simulink model "fft_4ch_nofir"  (R2012b)
settings: Solver=FixedStepDiscrete  SolverMode=SingleTasking  StartTime=0.0  StopTime=32768*5  FixedStep=0.25  RelTol=1e-3
libraries: xbsIndex_r4 x17003, casper_library_misc x133, casper_library_multipliers x20, casper_library_delays x19, xps_library x5, dspsrcs4 x3, xbsReplacements_r4 x2, simulink x1
(part 3 of 170)

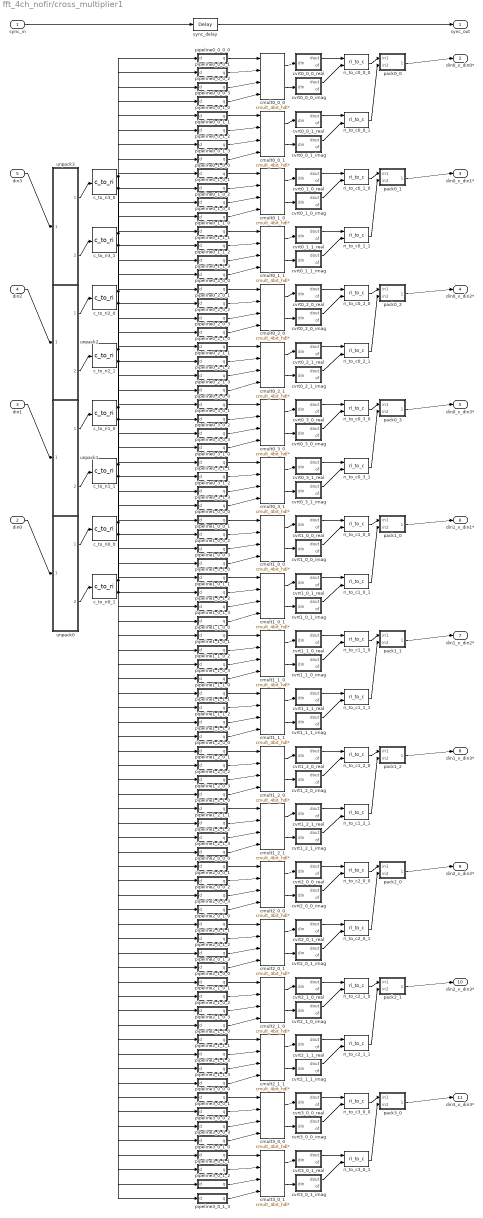
== system fft_4ch_nofir/cross_multiplier1 ==
  sync_in : Inport
  din0 : Inport  Port=2
  din1 : Inport  Port=3
  din2 : Inport  Port=4
  din3 : Inport  Port=5
  c_to_ri0_0 : casper_library_misc/c_to_ri  n_bits=bit_width_in  bin_pt=binary_point_in
  c_to_ri0_1 : casper_library_misc/c_to_ri  n_bits=bit_width_in  bin_pt=binary_point_in
  c_to_ri1_0 : casper_library_misc/c_to_ri  n_bits=bit_width_in  bin_pt=binary_point_in
  c_to_ri1_1 : casper_library_misc/c_to_ri  n_bits=bit_width_in  bin_pt=binary_point_in
  c_to_ri2_0 : casper_library_misc/c_to_ri  n_bits=bit_width_in  bin_pt=binary_point_in
  c_to_ri2_1 : casper_library_misc/c_to_ri  n_bits=bit_width_in  bin_pt=binary_point_in
  c_to_ri3_0 : casper_library_misc/c_to_ri  n_bits=bit_width_in  bin_pt=binary_point_in
  c_to_ri3_1 : casper_library_misc/c_to_ri  n_bits=bit_width_in  bin_pt=binary_point_in
  cmult0_0_0 : casper_library_multipliers/cmult_4bit_hdl*  mult_latency=mult_latency  add_latency=add_latency
      link override imag_sum: mode=Subtraction  use_carryin=off  use_carryout=off  en=off  latency=add_latency  precision=Full  arith_type=Unsigned  n_bits=8  bin_pt=2  quantization=Truncate  overflow=Wrap  dbl_ovrd=off  use_behavioral_HDL=on  hw_selection=Fabric  pipelined=off  use_rpm=on
      link override real_sum: mode=Addition  use_carryin=off  use_carryout=off  en=off  latency=add_latency  precision=Full  arith_type=Unsigned  n_bits=8  bin_pt=2  quantization=Truncate  overflow=Wrap  dbl_ovrd=off  use_behavioral_HDL=on  hw_selection=Fabric  pipelined=off  use_rpm=on
      link override imag_sum: xl_area=[4 8 0 7 0 0 0]
      link override real_sum: xl_area=[4 8 0 7 0 0 0]
  cmult0_0_1 : casper_library_multipliers/cmult_4bit_hdl*  mult_latency=mult_latency  add_latency=add_latency
  cmult0_1_0 : casper_library_multipliers/cmult_4bit_hdl*  mult_latency=mult_latency  add_latency=add_latency
  cmult0_1_1 : casper_library_multipliers/cmult_4bit_hdl*  mult_latency=mult_latency  add_latency=add_latency
  cmult0_2_0 : casper_library_multipliers/cmult_4bit_hdl*  mult_latency=mult_latency  add_latency=add_latency
  cmult0_2_1 : casper_library_multipliers/cmult_4bit_hdl*  mult_latency=mult_latency  add_latency=add_latency
  cmult0_3_0 : casper_library_multipliers/cmult_4bit_hdl*  mult_latency=mult_latency  add_latency=add_latency
  cmult0_3_1 : casper_library_multipliers/cmult_4bit_hdl*  mult_latency=mult_latency  add_latency=add_latency
  cmult1_0_0 : casper_library_multipliers/cmult_4bit_hdl*  mult_latency=mult_latency  add_latency=add_latency
  cmult1_0_1 : casper_library_multipliers/cmult_4bit_hdl*  mult_latency=mult_latency  add_latency=add_latency
  cmult1_1_0 : casper_library_multipliers/cmult_4bit_hdl*  mult_latency=mult_latency  add_latency=add_latency
  cmult1_1_1 : casper_library_multipliers/cmult_4bit_hdl*  mult_latency=mult_latency  add_latency=add_latency
  cmult1_2_0 : casper_library_multipliers/cmult_4bit_hdl*  mult_latency=mult_latency  add_latency=add_latency
  cmult1_2_1 : casper_library_multipliers/cmult_4bit_hdl*  mult_latency=mult_latency  add_latency=add_latency
  cmult2_0_0 : casper_library_multipliers/cmult_4bit_hdl*  mult_latency=mult_latency  add_latency=add_latency
  cmult2_0_1 : casper_library_multipliers/cmult_4bit_hdl*  mult_latency=mult_latency  add_latency=add_latency
  cmult2_1_0 : casper_library_multipliers/cmult_4bit_hdl*  mult_latency=mult_latency  add_latency=add_latency
  cmult2_1_1 : casper_library_multipliers/cmult_4bit_hdl*  mult_latency=mult_latency  add_latency=add_latency
  cmult3_0_0 : casper_library_multipliers/cmult_4bit_hdl*  mult_latency=mult_latency  add_latency=add_latency
  cmult3_0_1 : casper_library_multipliers/cmult_4bit_hdl*  mult_latency=mult_latency  add_latency=add_latency
  cvrt0_0_0_imag : Subsystem  AncestorBlock=casper_library_misc/convert_of  mask(convert_of){bit_width_i=37, binary_point_i=34, bit_width_o=37, binary_point_o=34, latency=0, overflow=Wrap, quantization=Truncate}
      mask prompts: bit_width_i "Bit Width In"; binary_point_i "Binary Point In"; bit_width_o "Bit Width Out"; binary_point_o "Binary Point Out"; overflow "Overflow Behaviour"; quantization "Quantization Behaviour"
      mask help:
      | Converts from one 2's complement bit-width
      | and/or binary point position to another.
      | Includes underflow/overflow indicator.
      mask init:
      | convert_of_init(gcb, ...
      |     'bit_width_i', bit_width_i, ...
      |     'binary_point_i', binary_point_i, ...
      |     'bit_width_o', bit_width_o, ...
      |     'binary_point_o', binary_point_o, ...
      |     'latency', latency, ...
      |     'overflow', overflow, ...
      |     'quantization', quantization);
      settings: AttributesFormatString=[37,34]->[37,34]
      mask TypeOptions overflow: Wrap | Saturate | Error
      mask TypeOptions quantization: Truncate | Round  (unbiased: +/- Inf) | Round  (unbiased: even values)
  cvrt0_0_0_real : Subsystem  AncestorBlock=casper_library_misc/convert_of  mask(convert_of){bit_width_i=37, binary_point_i=34, bit_width_o=37, binary_point_o=34, latency=0, overflow=Wrap, quantization=Truncate}
      mask prompts: bit_width_i "Bit Width In"; binary_point_i "Binary Point In"; bit_width_o "Bit Width Out"; binary_point_o "Binary Point Out"; overflow "Overflow Behaviour"; quantization "Quantization Behaviour"
      mask help:
      | Converts from one 2's complement bit-width
      | and/or binary point position to another.
      | Includes underflow/overflow indicator.
      mask init: same as fft_4ch_nofir/cross_multiplier1/cvrt0_0_0_imag
      settings: AttributesFormatString=[37,34]->[37,34]
      mask TypeOptions overflow: Wrap | Saturate | Error
      mask TypeOptions quantization: Truncate | Round  (unbiased: +/- Inf) | Round  (unbiased: even values)
  cvrt0_0_1_imag : Subsystem  AncestorBlock=casper_library_misc/convert_of  mask(convert_of){bit_width_i=37, binary_point_i=34, bit_width_o=37, binary_point_o=34, latency=0, overflow=Wrap, quantization=Truncate}
      mask prompts: bit_width_i "Bit Width In"; binary_point_i "Binary Point In"; bit_width_o "Bit Width Out"; binary_point_o "Binary Point Out"; overflow "Overflow Behaviour"; quantization "Quantization Behaviour"
      mask help:
      | Converts from one 2's complement bit-width
      | and/or binary point position to another.
      | Includes underflow/overflow indicator.
      mask init: same as fft_4ch_nofir/cross_multiplier1/cvrt0_0_0_imag
      settings: AttributesFormatString=[37,34]->[37,34]
      mask TypeOptions overflow: Wrap | Saturate | Error
      mask TypeOptions quantization: Truncate | Round  (unbiased: +/- Inf) | Round  (unbiased: even values)
  cvrt0_0_1_real : Subsystem  AncestorBlock=casper_library_misc/convert_of  mask(convert_of){bit_width_i=37, binary_point_i=34, bit_width_o=37, binary_point_o=34, latency=0, overflow=Wrap, quantization=Truncate}
      mask prompts: bit_width_i "Bit Width In"; binary_point_i "Binary Point In"; bit_width_o "Bit Width Out"; binary_point_o "Binary Point Out"; overflow "Overflow Behaviour"; quantization "Quantization Behaviour"
      mask help:
      | Converts from one 2's complement bit-width
      | and/or binary point position to another.
      | Includes underflow/overflow indicator.
      mask init: same as fft_4ch_nofir/cross_multiplier1/cvrt0_0_0_imag
      settings: AttributesFormatString=[37,34]->[37,34]
      mask TypeOptions overflow: Wrap | Saturate | Error
      mask TypeOptions quantization: Truncate | Round  (unbiased: +/- Inf) | Round  (unbiased: even values)
  cvrt0_1_0_imag : Subsystem  AncestorBlock=casper_library_misc/convert_of  mask(convert_of){bit_width_i=37, binary_point_i=34, bit_width_o=37, binary_point_o=34, latency=0, overflow=Wrap, quantization=Truncate}
      mask prompts: bit_width_i "Bit Width In"; binary_point_i "Binary Point In"; bit_width_o "Bit Width Out"; binary_point_o "Binary Point Out"; overflow "Overflow Behaviour"; quantization "Quantization Behaviour"
      mask help:
      | Converts from one 2's complement bit-width
      | and/or binary point position to another.
      | Includes underflow/overflow indicator.
      mask init: same as fft_4ch_nofir/cross_multiplier1/cvrt0_0_0_imag
      settings: AttributesFormatString=[37,34]->[37,34]
      mask TypeOptions overflow: Wrap | Saturate | Error
      mask TypeOptions quantization: Truncate | Round  (unbiased: +/- Inf) | Round  (unbiased: even values)
  cvrt0_1_0_real : Subsystem  AncestorBlock=casper_library_misc/convert_of  mask(convert_of){bit_width_i=37, binary_point_i=34, bit_width_o=37, binary_point_o=34, latency=0, overflow=Wrap, quantization=Truncate}
      mask prompts: bit_width_i "Bit Width In"; binary_point_i "Binary Point In"; bit_width_o "Bit Width Out"; binary_point_o "Binary Point Out"; overflow "Overflow Behaviour"; quantization "Quantization Behaviour"
      mask help:
      | Converts from one 2's complement bit-width
      | and/or binary point position to another.
      | Includes underflow/overflow indicator.
      mask init: same as fft_4ch_nofir/cross_multiplier1/cvrt0_0_0_imag
      settings: AttributesFormatString=[37,34]->[37,34]
      mask TypeOptions overflow: Wrap | Saturate | Error
      mask TypeOptions quantization: Truncate | Round  (unbiased: +/- Inf) | Round  (unbiased: even values)
  cvrt0_1_1_imag : Subsystem  AncestorBlock=casper_library_misc/convert_of  mask(convert_of){bit_width_i=37, binary_point_i=34, bit_width_o=37, binary_point_o=34, latency=0, overflow=Wrap, quantization=Truncate}
      mask prompts: bit_width_i "Bit Width In"; binary_point_i "Binary Point In"; bit_width_o "Bit Width Out"; binary_point_o "Binary Point Out"; overflow "Overflow Behaviour"; quantization "Quantization Behaviour"
      mask help:
      | Converts from one 2's complement bit-width
      | and/or binary point position to another.
      | Includes underflow/overflow indicator.
      mask init: same as fft_4ch_nofir/cross_multiplier1/cvrt0_0_0_imag
      settings: AttributesFormatString=[37,34]->[37,34]
      mask TypeOptions overflow: Wrap | Saturate | Error
      mask TypeOptions quantization: Truncate | Round  (unbiased: +/- Inf) | Round  (unbiased: even values)
  cvrt0_1_1_real : Subsystem  AncestorBlock=casper_library_misc/convert_of  mask(convert_of){bit_width_i=37, binary_point_i=34, bit_width_o=37, binary_point_o=34, latency=0, overflow=Wrap, quantization=Truncate}
      mask prompts: bit_width_i "Bit Width In"; binary_point_i "Binary Point In"; bit_width_o "Bit Width Out"; binary_point_o "Binary Point Out"; overflow "Overflow Behaviour"; quantization "Quantization Behaviour"
      mask help:
      | Converts from one 2's complement bit-width
      | and/or binary point position to another.
      | Includes underflow/overflow indicator.
      mask init: same as fft_4ch_nofir/cross_multiplier1/cvrt0_0_0_imag
      settings: AttributesFormatString=[37,34]->[37,34]
      mask TypeOptions overflow: Wrap | Saturate | Error
      mask TypeOptions quantization: Truncate | Round  (unbiased: +/- Inf) | Round  (unbiased: even values)
  cvrt0_2_0_imag : Subsystem  AncestorBlock=casper_library_misc/convert_of  mask(convert_of){bit_width_i=37, binary_point_i=34, bit_width_o=37, binary_point_o=34, latency=0, overflow=Wrap, quantization=Truncate}
      mask prompts: bit_width_i "Bit Width In"; binary_point_i "Binary Point In"; bit_width_o "Bit Width Out"; binary_point_o "Binary Point Out"; overflow "Overflow Behaviour"; quantization "Quantization Behaviour"
      mask help:
      | Converts from one 2's complement bit-width
      | and/or binary point position to another.
      | Includes underflow/overflow indicator.
      mask init: same as fft_4ch_nofir/cross_multiplier1/cvrt0_0_0_imag
      settings: AttributesFormatString=[37,34]->[37,34]
      mask TypeOptions overflow: Wrap | Saturate | Error
      mask TypeOptions quantization: Truncate | Round  (unbiased: +/- Inf) | Round  (unbiased: even values)
  cvrt0_2_0_real : Subsystem  AncestorBlock=casper_library_misc/convert_of  mask(convert_of){bit_width_i=37, binary_point_i=34, bit_width_o=37, binary_point_o=34, latency=0, overflow=Wrap, quantization=Truncate}
      mask prompts: bit_width_i "Bit Width In"; binary_point_i "Binary Point In"; bit_width_o "Bit Width Out"; binary_point_o "Binary Point Out"; overflow "Overflow Behaviour"; quantization "Quantization Behaviour"
      mask help:
      | Converts from one 2's complement bit-width
      | and/or binary point position to another.
      | Includes underflow/overflow indicator.
      mask init: same as fft_4ch_nofir/cross_multiplier1/cvrt0_0_0_imag
      settings: AttributesFormatString=[37,34]->[37,34]
      mask TypeOptions overflow: Wrap | Saturate | Error
      mask TypeOptions quantization: Truncate | Round  (unbiased: +/- Inf) | Round  (unbiased: even values)
  cvrt0_2_1_imag : Subsystem  AncestorBlock=casper_library_misc/convert_of  mask(convert_of){bit_width_i=37, binary_point_i=34, bit_width_o=37, binary_point_o=34, latency=0, overflow=Wrap, quantization=Truncate}
      mask prompts: bit_width_i "Bit Width In"; binary_point_i "Binary Point In"; bit_width_o "Bit Width Out"; binary_point_o "Binary Point Out"; overflow "Overflow Behaviour"; quantization "Quantization Behaviour"
      mask help:
      | Converts from one 2's complement bit-width
      | and/or binary point position to another.
      | Includes underflow/overflow indicator.
      mask init: same as fft_4ch_nofir/cross_multiplier1/cvrt0_0_0_imag
      settings: AttributesFormatString=[37,34]->[37,34]
      mask TypeOptions overflow: Wrap | Saturate | Error
      mask TypeOptions quantization: Truncate | Round  (unbiased: +/- Inf) | Round  (unbiased: even values)
  cvrt0_2_1_real : Subsystem  AncestorBlock=casper_library_misc/convert_of  mask(convert_of){bit_width_i=37, binary_point_i=34, bit_width_o=37, binary_point_o=34, latency=0, overflow=Wrap, quantization=Truncate}
      mask prompts: bit_width_i "Bit Width In"; binary_point_i "Binary Point In"; bit_width_o "Bit Width Out"; binary_point_o "Binary Point Out"; overflow "Overflow Behaviour"; quantization "Quantization Behaviour"
      mask help:
      | Converts from one 2's complement bit-width
      | and/or binary point position to another.
      | Includes underflow/overflow indicator.
      mask init: same as fft_4ch_nofir/cross_multiplier1/cvrt0_0_0_imag
      settings: AttributesFormatString=[37,34]->[37,34]
      mask TypeOptions overflow: Wrap | Saturate | Error
      mask TypeOptions quantization: Truncate | Round  (unbiased: +/- Inf) | Round  (unbiased: even values)
  cvrt0_3_0_imag : Subsystem  AncestorBlock=casper_library_misc/convert_of  mask(convert_of){bit_width_i=37, binary_point_i=34, bit_width_o=37, binary_point_o=34, latency=0, overflow=Wrap, quantization=Truncate}
      mask prompts: bit_width_i "Bit Width In"; binary_point_i "Binary Point In"; bit_width_o "Bit Width Out"; binary_point_o "Binary Point Out"; overflow "Overflow Behaviour"; quantization "Quantization Behaviour"
      mask help:
      | Converts from one 2's complement bit-width
      | and/or binary point position to another.
      | Includes underflow/overflow indicator.
      mask init: same as fft_4ch_nofir/cross_multiplier1/cvrt0_0_0_imag
      settings: AttributesFormatString=[37,34]->[37,34]
      mask TypeOptions overflow: Wrap | Saturate | Error
      mask TypeOptions quantization: Truncate | Round  (unbiased: +/- Inf) | Round  (unbiased: even values)
  cvrt0_3_0_real : Subsystem  AncestorBlock=casper_library_misc/convert_of  mask(convert_of){bit_width_i=37, binary_point_i=34, bit_width_o=37, binary_point_o=34, latency=0, overflow=Wrap, quantization=Truncate}
      mask prompts: bit_width_i "Bit Width In"; binary_point_i "Binary Point In"; bit_width_o "Bit Width Out"; binary_point_o "Binary Point Out"; overflow "Overflow Behaviour"; quantization "Quantization Behaviour"
      mask help:
      | Converts from one 2's complement bit-width
      | and/or binary point position to another.
      | Includes underflow/overflow indicator.
      mask init: same as fft_4ch_nofir/cross_multiplier1/cvrt0_0_0_imag
      settings: AttributesFormatString=[37,34]->[37,34]
      mask TypeOptions overflow: Wrap | Saturate | Error
      mask TypeOptions quantization: Truncate | Round  (unbiased: +/- Inf) | Round  (unbiased: even values)
  cvrt0_3_1_imag : Subsystem  AncestorBlock=casper_library_misc/convert_of  mask(convert_of){bit_width_i=37, binary_point_i=34, bit_width_o=37, binary_point_o=34, latency=0, overflow=Wrap, quantization=Truncate}
      mask prompts: bit_width_i "Bit Width In"; binary_point_i "Binary Point In"; bit_width_o "Bit Width Out"; binary_point_o "Binary Point Out"; overflow "Overflow Behaviour"; quantization "Quantization Behaviour"
      mask help:
      | Converts from one 2's complement bit-width
      | and/or binary point position to another.
      | Includes underflow/overflow indicator.
      mask init: same as fft_4ch_nofir/cross_multiplier1/cvrt0_0_0_imag
      settings: AttributesFormatString=[37,34]->[37,34]
      mask TypeOptions overflow: Wrap | Saturate | Error
      mask TypeOptions quantization: Truncate | Round  (unbiased: +/- Inf) | Round  (unbiased: even values)
  cvrt0_3_1_real : Subsystem  AncestorBlock=casper_library_misc/convert_of  mask(convert_of){bit_width_i=37, binary_point_i=34, bit_width_o=37, binary_point_o=34, latency=0, overflow=Wrap, quantization=Truncate}
      mask prompts: bit_width_i "Bit Width In"; binary_point_i "Binary Point In"; bit_width_o "Bit Width Out"; binary_point_o "Binary Point Out"; overflow "Overflow Behaviour"; quantization "Quantization Behaviour"
      mask help:
      | Converts from one 2's complement bit-width
      | and/or binary point position to another.
      | Includes underflow/overflow indicator.
      mask init: same as fft_4ch_nofir/cross_multiplier1/cvrt0_0_0_imag
      settings: AttributesFormatString=[37,34]->[37,34]
      mask TypeOptions overflow: Wrap | Saturate | Error
      mask TypeOptions quantization: Truncate | Round  (unbiased: +/- Inf) | Round  (unbiased: even values)
  cvrt1_0_0_imag : Subsystem  AncestorBlock=casper_library_misc/convert_of  mask(convert_of){bit_width_i=37, binary_point_i=34, bit_width_o=37, binary_point_o=34, latency=0, overflow=Wrap, quantization=Truncate}
      mask prompts: bit_width_i "Bit Width In"; binary_point_i "Binary Point In"; bit_width_o "Bit Width Out"; binary_point_o "Binary Point Out"; overflow "Overflow Behaviour"; quantization "Quantization Behaviour"
      mask help:
      | Converts from one 2's complement bit-width
      | and/or binary point position to another.
      | Includes underflow/overflow indicator.
      mask init: same as fft_4ch_nofir/cross_multiplier1/cvrt0_0_0_imag
      settings: AttributesFormatString=[37,34]->[37,34]
      mask TypeOptions overflow: Wrap | Saturate | Error
      mask TypeOptions quantization: Truncate | Round  (unbiased: +/- Inf) | Round  (unbiased: even values)
  cvrt1_0_0_real : Subsystem  AncestorBlock=casper_library_misc/convert_of  mask(convert_of){bit_width_i=37, binary_point_i=34, bit_width_o=37, binary_point_o=34, latency=0, overflow=Wrap, quantization=Truncate}
      mask prompts: bit_width_i "Bit Width In"; binary_point_i "Binary Point In"; bit_width_o "Bit Width Out"; binary_point_o "Binary Point Out"; overflow "Overflow Behaviour"; quantization "Quantization Behaviour"
      mask help:
      | Converts from one 2's complement bit-width
      | and/or binary point position to another.
      | Includes underflow/overflow indicator.
      mask init: same as fft_4ch_nofir/cross_multiplier1/cvrt0_0_0_imag
      settings: AttributesFormatString=[37,34]->[37,34]
      mask TypeOptions overflow: Wrap | Saturate | Error
      mask TypeOptions quantization: Truncate | Round  (unbiased: +/- Inf) | Round  (unbiased: even values)
  cvrt1_0_1_imag : Subsystem  AncestorBlock=casper_library_misc/convert_of  mask(convert_of){bit_width_i=37, binary_point_i=34, bit_width_o=37, binary_point_o=34, latency=0, overflow=Wrap, quantization=Truncate}
      mask prompts: bit_width_i "Bit Width In"; binary_point_i "Binary Point In"; bit_width_o "Bit Width Out"; binary_point_o "Binary Point Out"; overflow "Overflow Behaviour"; quantization "Quantization Behaviour"
      mask help:
      | Converts from one 2's complement bit-width
      | and/or binary point position to another.
      | Includes underflow/overflow indicator.
      mask init: same as fft_4ch_nofir/cross_multiplier1/cvrt0_0_0_imag
      settings: AttributesFormatString=[37,34]->[37,34]
      mask TypeOptions overflow: Wrap | Saturate | Error
      mask TypeOptions quantization: Truncate | Round  (unbiased: +/- Inf) | Round  (unbiased: even values)
  cvrt1_0_1_real : Subsystem  AncestorBlock=casper_library_misc/convert_of  mask(convert_of){bit_width_i=37, binary_point_i=34, bit_width_o=37, binary_point_o=34, latency=0, overflow=Wrap, quantization=Truncate}
      mask prompts: bit_width_i "Bit Width In"; binary_point_i "Binary Point In"; bit_width_o "Bit Width Out"; binary_point_o "Binary Point Out"; overflow "Overflow Behaviour"; quantization "Quantization Behaviour"
      mask help:
      | Converts from one 2's complement bit-width
      | and/or binary point position to another.
      | Includes underflow/overflow indicator.
      mask init: same as fft_4ch_nofir/cross_multiplier1/cvrt0_0_0_imag
      settings: AttributesFormatString=[37,34]->[37,34]
      mask TypeOptions overflow: Wrap | Saturate | Error
      mask TypeOptions quantization: Truncate | Round  (unbiased: +/- Inf) | Round  (unbiased: even values)
  cvrt1_1_0_imag : Subsystem  AncestorBlock=casper_library_misc/convert_of  mask(convert_of){bit_width_i=37, binary_point_i=34, bit_width_o=37, binary_point_o=34, latency=0, overflow=Wrap, quantization=Truncate}
      mask prompts: bit_width_i "Bit Width In"; binary_point_i "Binary Point In"; bit_width_o "Bit Width Out"; binary_point_o "Binary Point Out"; overflow "Overflow Behaviour"; quantization "Quantization Behaviour"
      mask help:
      | Converts from one 2's complement bit-width
      | and/or binary point position to another.
      | Includes underflow/overflow indicator.
      mask init: same as fft_4ch_nofir/cross_multiplier1/cvrt0_0_0_imag
      settings: AttributesFormatString=[37,34]->[37,34]
      mask TypeOptions overflow: Wrap | Saturate | Error
      mask TypeOptions quantization: Truncate | Round  (unbiased: +/- Inf) | Round  (unbiased: even values)
  cvrt1_1_0_real : Subsystem  AncestorBlock=casper_library_misc/convert_of  mask(convert_of){bit_width_i=37, binary_point_i=34, bit_width_o=37, binary_point_o=34, latency=0, overflow=Wrap, quantization=Truncate}
      mask prompts: bit_width_i "Bit Width In"; binary_point_i "Binary Point In"; bit_width_o "Bit Width Out"; binary_point_o "Binary Point Out"; overflow "Overflow Behaviour"; quantization "Quantization Behaviour"
      mask help:
      | Converts from one 2's complement bit-width
      | and/or binary point position to another.
      | Includes underflow/overflow indicator.
      mask init: same as fft_4ch_nofir/cross_multiplier1/cvrt0_0_0_imag
      settings: AttributesFormatString=[37,34]->[37,34]
      mask TypeOptions overflow: Wrap | Saturate | Error
      mask TypeOptions quantization: Truncate | Round  (unbiased: +/- Inf) | Round  (unbiased: even values)
  cvrt1_1_1_imag : Subsystem  AncestorBlock=casper_library_misc/convert_of  mask(convert_of){bit_width_i=37, binary_point_i=34, bit_width_o=37, binary_point_o=34, latency=0, overflow=Wrap, quantization=Truncate}
      mask prompts: bit_width_i "Bit Width In"; binary_point_i "Binary Point In"; bit_width_o "Bit Width Out"; binary_point_o "Binary Point Out"; overflow "Overflow Behaviour"; quantization "Quantization Behaviour"
      mask help:
      | Converts from one 2's complement bit-width
      | and/or binary point position to another.
      | Includes underflow/overflow indicator.
      mask init: same as fft_4ch_nofir/cross_multiplier1/cvrt0_0_0_imag
      settings: AttributesFormatString=[37,34]->[37,34]
      mask TypeOptions overflow: Wrap | Saturate | Error
      mask TypeOptions quantization: Truncate | Round  (unbiased: +/- Inf) | Round  (unbiased: even values)
  cvrt1_1_1_real : Subsystem  AncestorBlock=casper_library_misc/convert_of  mask(convert_of){bit_width_i=37, binary_point_i=34, bit_width_o=37, binary_point_o=34, latency=0, overflow=Wrap, quantization=Truncate}
      mask prompts: bit_width_i "Bit Width In"; binary_point_i "Binary Point In"; bit_width_o "Bit Width Out"; binary_point_o "Binary Point Out"; overflow "Overflow Behaviour"; quantization "Quantization Behaviour"
      mask help:
      | Converts from one 2's complement bit-width
      | and/or binary point position to another.
      | Includes underflow/overflow indicator.
      mask init: same as fft_4ch_nofir/cross_multiplier1/cvrt0_0_0_imag
      settings: AttributesFormatString=[37,34]->[37,34]
      mask TypeOptions overflow: Wrap | Saturate | Error
      mask TypeOptions quantization: Truncate | Round  (unbiased: +/- Inf) | Round  (unbiased: even values)
  cvrt1_2_0_imag : Subsystem  AncestorBlock=casper_library_misc/convert_of  mask(convert_of){bit_width_i=37, binary_point_i=34, bit_width_o=37, binary_point_o=34, latency=0, overflow=Wrap, quantization=Truncate}
      mask prompts: bit_width_i "Bit Width In"; binary_point_i "Binary Point In"; bit_width_o "Bit Width Out"; binary_point_o "Binary Point Out"; overflow "Overflow Behaviour"; quantization "Quantization Behaviour"
      mask help:
      | Converts from one 2's complement bit-width
      | and/or binary point position to another.
      | Includes underflow/overflow indicator.
      mask init: same as fft_4ch_nofir/cross_multiplier1/cvrt0_0_0_imag
      settings: AttributesFormatString=[37,34]->[37,34]
      mask TypeOptions overflow: Wrap | Saturate | Error
      mask TypeOptions quantization: Truncate | Round  (unbiased: +/- Inf) | Round  (unbiased: even values)
  cvrt1_2_0_real : Subsystem  AncestorBlock=casper_library_misc/convert_of  mask(convert_of){bit_width_i=37, binary_point_i=34, bit_width_o=37, binary_point_o=34, latency=0, overflow=Wrap, quantization=Truncate}
      mask prompts: bit_width_i "Bit Width In"; binary_point_i "Binary Point In"; bit_width_o "Bit Width Out"; binary_point_o "Binary Point Out"; overflow "Overflow Behaviour"; quantization "Quantization Behaviour"
      mask help:
      | Converts from one 2's complement bit-width
      | and/or binary point position to another.
      | Includes underflow/overflow indicator.
      mask init: same as fft_4ch_nofir/cross_multiplier1/cvrt0_0_0_imag
      settings: AttributesFormatString=[37,34]->[37,34]
      mask TypeOptions overflow: Wrap | Saturate | Error
      mask TypeOptions quantization: Truncate | Round  (unbiased: +/- Inf) | Round  (unbiased: even values)
  cvrt1_2_1_imag : Subsystem  AncestorBlock=casper_library_misc/convert_of  mask(convert_of){bit_width_i=37, binary_point_i=34, bit_width_o=37, binary_point_o=34, latency=0, overflow=Wrap, quantization=Truncate}
      mask prompts: bit_width_i "Bit Width In"; binary_point_i "Binary Point In"; bit_width_o "Bit Width Out"; binary_point_o "Binary Point Out"; overflow "Overflow Behaviour"; quantization "Quantization Behaviour"
      mask help:
      | Converts from one 2's complement bit-width
      | and/or binary point position to another.
      | Includes underflow/overflow indicator.
      mask init: same as fft_4ch_nofir/cross_multiplier1/cvrt0_0_0_imag
      settings: AttributesFormatString=[37,34]->[37,34]
      mask TypeOptions overflow: Wrap | Saturate | Error
      mask TypeOptions quantization: Truncate | Round  (unbiased: +/- Inf) | Round  (unbiased: even values)
  cvrt1_2_1_real : Subsystem  AncestorBlock=casper_library_misc/convert_of  mask(convert_of){bit_width_i=37, binary_point_i=34, bit_width_o=37, binary_point_o=34, latency=0, overflow=Wrap, quantization=Truncate}
      mask prompts: bit_width_i "Bit Width In"; binary_point_i "Binary Point In"; bit_width_o "Bit Width Out"; binary_point_o "Binary Point Out"; overflow "Overflow Behaviour"; quantization "Quantization Behaviour"
      mask help:
      | Converts from one 2's complement bit-width
      | and/or binary point position to another.
      | Includes underflow/overflow indicator.
      mask init: same as fft_4ch_nofir/cross_multiplier1/cvrt0_0_0_imag
      settings: AttributesFormatString=[37,34]->[37,34]
      mask TypeOptions overflow: Wrap | Saturate | Error
      mask TypeOptions quantization: Truncate | Round  (unbiased: +/- Inf) | Round  (unbiased: even values)
  cvrt2_0_0_imag : Subsystem  AncestorBlock=casper_library_misc/convert_of  mask(convert_of){bit_width_i=37, binary_point_i=34, bit_width_o=37, binary_point_o=34, latency=0, overflow=Wrap, quantization=Truncate}
      mask prompts: bit_width_i "Bit Width In"; binary_point_i "Binary Point In"; bit_width_o "Bit Width Out"; binary_point_o "Binary Point Out"; overflow "Overflow Behaviour"; quantization "Quantization Behaviour"
      mask help:
      | Converts from one 2's complement bit-width
      | and/or binary point position to another.
      | Includes underflow/overflow indicator.
      mask init: same as fft_4ch_nofir/cross_multiplier1/cvrt0_0_0_imag
      settings: AttributesFormatString=[37,34]->[37,34]
      mask TypeOptions overflow: Wrap | Saturate | Error
      mask TypeOptions quantization: Truncate | Round  (unbiased: +/- Inf) | Round  (unbiased: even values)
  cvrt2_0_0_real : Subsystem  AncestorBlock=casper_library_misc/convert_of  mask(convert_of){bit_width_i=37, binary_point_i=34, bit_width_o=37, binary_point_o=34, latency=0, overflow=Wrap, quantization=Truncate}
      mask prompts: bit_width_i "Bit Width In"; binary_point_i "Binary Point In"; bit_width_o "Bit Width Out"; binary_point_o "Binary Point Out"; overflow "Overflow Behaviour"; quantization "Quantization Behaviour"
      mask help:
      | Converts from one 2's complement bit-width
      | and/or binary point position to another.
      | Includes underflow/overflow indicator.
      mask init: same as fft_4ch_nofir/cross_multiplier1/cvrt0_0_0_imag
      settings: AttributesFormatString=[37,34]->[37,34]
      mask TypeOptions overflow: Wrap | Saturate | Error
      mask TypeOptions quantization: Truncate | Round  (unbiased: +/- Inf) | Round  (unbiased: even values)
  cvrt2_0_1_imag : Subsystem  AncestorBlock=casper_library_misc/convert_of  mask(convert_of){bit_width_i=37, binary_point_i=34, bit_width_o=37, binary_point_o=34, latency=0, overflow=Wrap, quantization=Truncate}
      mask prompts: bit_width_i "Bit Width In"; binary_point_i "Binary Point In"; bit_width_o "Bit Width Out"; binary_point_o "Binary Point Out"; overflow "Overflow Behaviour"; quantization "Quantization Behaviour"
      mask help:
      | Converts from one 2's complement bit-width
      | and/or binary point position to another.
      | Includes underflow/overflow indicator.
      mask init: same as fft_4ch_nofir/cross_multiplier1/cvrt0_0_0_imag
      settings: AttributesFormatString=[37,34]->[37,34]
      mask TypeOptions overflow: Wrap | Saturate | Error
      mask TypeOptions quantization: Truncate | Round  (unbiased: +/- Inf) | Round  (unbiased: even values)
  cvrt2_0_1_real : Subsystem  AncestorBlock=casper_library_misc/convert_of  mask(convert_of){bit_width_i=37, binary_point_i=34, bit_width_o=37, binary_point_o=34, latency=0, overflow=Wrap, quantization=Truncate}
      mask prompts: bit_width_i "Bit Width In"; binary_point_i "Binary Point In"; bit_width_o "Bit Width Out"; binary_point_o "Binary Point Out"; overflow "Overflow Behaviour"; quantization "Quantization Behaviour"
      mask help:
      | Converts from one 2's complement bit-width
      | and/or binary point position to another.
      | Includes underflow/overflow indicator.
      mask init: same as fft_4ch_nofir/cross_multiplier1/cvrt0_0_0_imag
      settings: AttributesFormatString=[37,34]->[37,34]
      mask TypeOptions overflow: Wrap | Saturate | Error
      mask TypeOptions quantization: Truncate | Round  (unbiased: +/- Inf) | Round  (unbiased: even values)
  cvrt2_1_0_imag : Subsystem  AncestorBlock=casper_library_misc/convert_of  mask(convert_of){bit_width_i=37, binary_point_i=34, bit_width_o=37, binary_point_o=34, latency=0, overflow=Wrap, quantization=Truncate}
      mask prompts: bit_width_i "Bit Width In"; binary_point_i "Binary Point In"; bit_width_o "Bit Width Out"; binary_point_o "Binary Point Out"; overflow "Overflow Behaviour"; quantization "Quantization Behaviour"
      mask help:
      | Converts from one 2's complement bit-width
      | and/or binary point position to another.
      | Includes underflow/overflow indicator.
      mask init: same as fft_4ch_nofir/cross_multiplier1/cvrt0_0_0_imag
      settings: AttributesFormatString=[37,34]->[37,34]
      mask TypeOptions overflow: Wrap | Saturate | Error
      mask TypeOptions quantization: Truncate | Round  (unbiased: +/- Inf) | Round  (unbiased: even values)
  cvrt2_1_0_real : Subsystem  AncestorBlock=casper_library_misc/convert_of  mask(convert_of){bit_width_i=37, binary_point_i=34, bit_width_o=37, binary_point_o=34, latency=0, overflow=Wrap, quantization=Truncate}
      mask prompts: bit_width_i "Bit Width In"; binary_point_i "Binary Point In"; bit_width_o "Bit Width Out"; binary_point_o "Binary Point Out"; overflow "Overflow Behaviour"; quantization "Quantization Behaviour"
      mask help:
      | Converts from one 2's complement bit-width
      | and/or binary point position to another.
      | Includes underflow/overflow indicator.
      mask init: same as fft_4ch_nofir/cross_multiplier1/cvrt0_0_0_imag
      settings: AttributesFormatString=[37,34]->[37,34]
      mask TypeOptions overflow: Wrap | Saturate | Error
      mask TypeOptions quantization: Truncate | Round  (unbiased: +/- Inf) | Round  (unbiased: even values)
  cvrt2_1_1_imag : Subsystem  AncestorBlock=casper_library_misc/convert_of  mask(convert_of){bit_width_i=37, binary_point_i=34, bit_width_o=37, binary_point_o=34, latency=0, overflow=Wrap, quantization=Truncate}
      mask prompts: bit_width_i "Bit Width In"; binary_point_i "Binary Point In"; bit_width_o "Bit Width Out"; binary_point_o "Binary Point Out"; overflow "Overflow Behaviour"; quantization "Quantization Behaviour"
      mask help:
      | Converts from one 2's complement bit-width
      | and/or binary point position to another.
      | Includes underflow/overflow indicator.
      mask init: same as fft_4ch_nofir/cross_multiplier1/cvrt0_0_0_imag
      settings: AttributesFormatString=[37,34]->[37,34]
      mask TypeOptions overflow: Wrap | Saturate | Error
      mask TypeOptions quantization: Truncate | Round  (unbiased: +/- Inf) | Round  (unbiased: even values)
  cvrt2_1_1_real : Subsystem  AncestorBlock=casper_library_misc/convert_of  mask(convert_of){bit_width_i=37, binary_point_i=34, bit_width_o=37, binary_point_o=34, latency=0, overflow=Wrap, quantization=Truncate}
      mask prompts: bit_width_i "Bit Width In"; binary_point_i "Binary Point In"; bit_width_o "Bit Width Out"; binary_point_o "Binary Point Out"; overflow "Overflow Behaviour"; quantization "Quantization Behaviour"
      mask help:
      | Converts from one 2's complement bit-width
      | and/or binary point position to another.
      | Includes underflow/overflow indicator.
      mask init: same as fft_4ch_nofir/cross_multiplier1/cvrt0_0_0_imag
      settings: AttributesFormatString=[37,34]->[37,34]
      mask TypeOptions overflow: Wrap | Saturate | Error
      mask TypeOptions quantization: Truncate | Round  (unbiased: +/- Inf) | Round  (unbiased: even values)
  cvrt3_0_0_imag : Subsystem  AncestorBlock=casper_library_misc/convert_of  mask(convert_of){bit_width_i=37, binary_point_i=34, bit_width_o=37, binary_point_o=34, latency=0, overflow=Wrap, quantization=Truncate}
      mask prompts: bit_width_i "Bit Width In"; binary_point_i "Binary Point In"; bit_width_o "Bit Width Out"; binary_point_o "Binary Point Out"; overflow "Overflow Behaviour"; quantization "Quantization Behaviour"
      mask help:
      | Converts from one 2's complement bit-width
      | and/or binary point position to another.
      | Includes underflow/overflow indicator.
      mask init: same as fft_4ch_nofir/cross_multiplier1/cvrt0_0_0_imag
      settings: AttributesFormatString=[37,34]->[37,34]
      mask TypeOptions overflow: Wrap | Saturate | Error
      mask TypeOptions quantization: Truncate | Round  (unbiased: +/- Inf) | Round  (unbiased: even values)
  cvrt3_0_0_real : Subsystem  AncestorBlock=casper_library_misc/convert_of  mask(convert_of){bit_width_i=37, binary_point_i=34, bit_width_o=37, binary_point_o=34, latency=0, overflow=Wrap, quantization=Truncate}
      mask prompts: bit_width_i "Bit Width In"; binary_point_i "Binary Point In"; bit_width_o "Bit Width Out"; binary_point_o "Binary Point Out"; overflow "Overflow Behaviour"; quantization "Quantization Behaviour"
      mask help:
      | Converts from one 2's complement bit-width
      | and/or binary point position to another.
      | Includes underflow/overflow indicator.
      mask init: same as fft_4ch_nofir/cross_multiplier1/cvrt0_0_0_imag
      settings: AttributesFormatString=[37,34]->[37,34]
      mask TypeOptions overflow: Wrap | Saturate | Error
      mask TypeOptions quantization: Truncate | Round  (unbiased: +/- Inf) | Round  (unbiased: even values)
  cvrt3_0_1_imag : Subsystem  AncestorBlock=casper_library_misc/convert_of  mask(convert_of){bit_width_i=37, binary_point_i=34, bit_width_o=37, binary_point_o=34, latency=0, overflow=Wrap, quantization=Truncate}
      mask prompts: bit_width_i "Bit Width In"; binary_point_i "Binary Point In"; bit_width_o "Bit Width Out"; binary_point_o "Binary Point Out"; overflow "Overflow Behaviour"; quantization "Quantization Behaviour"
      mask help:
      | Converts from one 2's complement bit-width
      | and/or binary point position to another.
      | Includes underflow/overflow indicator.
      mask init: same as fft_4ch_nofir/cross_multiplier1/cvrt0_0_0_imag
      settings: AttributesFormatString=[37,34]->[37,34]
      mask TypeOptions overflow: Wrap | Saturate | Error
      mask TypeOptions quantization: Truncate | Round  (unbiased: +/- Inf) | Round  (unbiased: even values)
  cvrt3_0_1_real : Subsystem  AncestorBlock=casper_library_misc/convert_of  mask(convert_of){bit_width_i=37, binary_point_i=34, bit_width_o=37, binary_point_o=34, latency=0, overflow=Wrap, quantization=Truncate}
      mask prompts: bit_width_i "Bit Width In"; binary_point_i "Binary Point In"; bit_width_o "Bit Width Out"; binary_point_o "Binary Point Out"; overflow "Overflow Behaviour"; quantization "Quantization Behaviour"
      mask help:
      | Converts from one 2's complement bit-width
      | and/or binary point position to another.
      | Includes underflow/overflow indicator.
      mask init: same as fft_4ch_nofir/cross_multiplier1/cvrt0_0_0_imag
      settings: AttributesFormatString=[37,34]->[37,34]
      mask TypeOptions overflow: Wrap | Saturate | Error
      mask TypeOptions quantization: Truncate | Round  (unbiased: +/- Inf) | Round  (unbiased: even values)
  pack0_0 : Subsystem  AncestorBlock=casper_library_flow_control/bus_create  mask(bus_create){inputNum=aggregation}
      mask prompts: inputNum "Number of inputs:"
      mask init:
      | bus_create_init(gcb,...
      |     'inputNum', inputNum);
  pack0_1 : Subsystem  AncestorBlock=casper_library_flow_control/bus_create  mask(bus_create){inputNum=aggregation}
      mask prompts: inputNum "Number of inputs:"
      mask init:
      | bus_create_init(gcb,...
      |     'inputNum', inputNum);
  pack0_2 : Subsystem  AncestorBlock=casper_library_flow_control/bus_create  mask(bus_create){inputNum=aggregation}
      mask prompts: inputNum "Number of inputs:"
      mask init:
      | bus_create_init(gcb,...
      |     'inputNum', inputNum);
  pack0_3 : Subsystem  AncestorBlock=casper_library_flow_control/bus_create  mask(bus_create){inputNum=aggregation}
      mask prompts: inputNum "Number of inputs:"
      mask init:
      | bus_create_init(gcb,...
      |     'inputNum', inputNum);
  pack1_0 : Subsystem  AncestorBlock=casper_library_flow_control/bus_create  mask(bus_create){inputNum=aggregation}
      mask prompts: inputNum "Number of inputs:"
      mask init:
      | bus_create_init(gcb,...
      |     'inputNum', inputNum);
  pack1_1 : Subsystem  AncestorBlock=casper_library_flow_control/bus_create  mask(bus_create){inputNum=aggregation}
      mask prompts: inputNum "Number of inputs:"
      mask init:
      | bus_create_init(gcb,...
      |     'inputNum', inputNum);
  pack1_2 : Subsystem  AncestorBlock=casper_library_flow_control/bus_create  mask(bus_create){inputNum=aggregation}
      mask prompts: inputNum "Number of inputs:"
      mask init:
      | bus_create_init(gcb,...
      |     'inputNum', inputNum);
  pack2_0 : Subsystem  AncestorBlock=casper_library_flow_control/bus_create  mask(bus_create){inputNum=aggregation}
      mask prompts: inputNum "Number of inputs:"
      mask init:
      | bus_create_init(gcb,...
      |     'inputNum', inputNum);
  pack2_1 : Subsystem  AncestorBlock=casper_library_flow_control/bus_create  mask(bus_create){inputNum=aggregation}
      mask prompts: inputNum "Number of inputs:"
      mask init:
      | bus_create_init(gcb,...
      |     'inputNum', inputNum);
  pack3_0 : Subsystem  AncestorBlock=casper_library_flow_control/bus_create  mask(bus_create){inputNum=aggregation}
      mask prompts: inputNum "Number of inputs:"
      mask init:
      | bus_create_init(gcb,...
      |     'inputNum', inputNum);
  pipeline0_0_0_0 : Subsystem  AncestorBlock=casper_library_delays/pipeline  mask(pipeline){latency=fanout_latency}
      mask help:
      | An explicitly laid-out delay line to avoid mapping to SRL16s
      | for use in pipelining to help achieve timing closure.
      mask init:
      | pipeline_init(gcb,'latency',latency);
      settings: AttributesFormatString=Latency = %<latency>
      mask Display:
      | port_label('input', 1, 'd');
      | port_label('output', 1, 'q');
      | disp(['Z^-', num2str(latency)]);
  pipeline0_0_0_1 : Subsystem  AncestorBlock=casper_library_delays/pipeline  mask(pipeline){latency=fanout_latency}
      mask help:
      | An explicitly laid-out delay line to avoid mapping to SRL16s
      | for use in pipelining to help achieve timing closure.
      mask init:
      | pipeline_init(gcb,'latency',latency);
      settings: AttributesFormatString=Latency = %<latency>
      mask Display:
      | port_label('input', 1, 'd');
      | port_label('output', 1, 'q');
      | disp(['Z^-', num2str(latency)]);
  pipeline0_0_0_2 : Subsystem  AncestorBlock=casper_library_delays/pipeline  mask(pipeline){latency=fanout_latency}
      mask help:
      | An explicitly laid-out delay line to avoid mapping to SRL16s
      | for use in pipelining to help achieve timing closure.
      mask init:
      | pipeline_init(gcb,'latency',latency);
      settings: AttributesFormatString=Latency = %<latency>
      mask Display:
      | port_label('input', 1, 'd');
      | port_label('output', 1, 'q');
      | disp(['Z^-', num2str(latency)]);
  pipeline0_0_0_3 : Subsystem  AncestorBlock=casper_library_delays/pipeline  mask(pipeline){latency=fanout_latency}
      mask help:
      | An explicitly laid-out delay line to avoid mapping to SRL16s
      | for use in pipelining to help achieve timing closure.
      mask init:
      | pipeline_init(gcb,'latency',latency);
      settings: AttributesFormatString=Latency = %<latency>
      mask Display:
      | port_label('input', 1, 'd');
      | port_label('output', 1, 'q');
      | disp(['Z^-', num2str(latency)]);
  pipeline0_0_1_0 : Subsystem  AncestorBlock=casper_library_delays/pipeline  mask(pipeline){latency=fanout_latency}
      mask help:
      | An explicitly laid-out delay line to avoid mapping to SRL16s
      | for use in pipelining to help achieve timing closure.
      mask init:
      | pipeline_init(gcb,'latency',latency);
      settings: AttributesFormatString=Latency = %<latency>
      mask Display:
      | port_label('input', 1, 'd');
      | port_label('output', 1, 'q');
      | disp(['Z^-', num2str(latency)]);
  pipeline0_0_1_1 : Subsystem  AncestorBlock=casper_library_delays/pipeline  mask(pipeline){latency=fanout_latency}
      mask help:
      | An explicitly laid-out delay line to avoid mapping to SRL16s
      | for use in pipelining to help achieve timing closure.
      mask init:
      | pipeline_init(gcb,'latency',latency);
      settings: AttributesFormatString=Latency = %<latency>
      mask Display:
      | port_label('input', 1, 'd');
      | port_label('output', 1, 'q');
      | disp(['Z^-', num2str(latency)]);
  pipeline0_0_1_2 : Subsystem  AncestorBlock=casper_library_delays/pipeline  mask(pipeline){latency=fanout_latency}
      mask help:
      | An explicitly laid-out delay line to avoid mapping to SRL16s
      | for use in pipelining to help achieve timing closure.
      mask init:
      | pipeline_init(gcb,'latency',latency);
      settings: AttributesFormatString=Latency = %<latency>
      mask Display:
      | port_label('input', 1, 'd');
      | port_label('output', 1, 'q');
      | disp(['Z^-', num2str(latency)]);
  pipeline0_0_1_3 : Subsystem  AncestorBlock=casper_library_delays/pipeline  mask(pipeline){latency=fanout_latency}
      mask help:
      | An explicitly laid-out delay line to avoid mapping to SRL16s
      | for use in pipelining to help achieve timing closure.
      mask init:
      | pipeline_init(gcb,'latency',latency);
      settings: AttributesFormatString=Latency = %<latency>
      mask Display:
      | port_label('input', 1, 'd');
      | port_label('output', 1, 'q');
      | disp(['Z^-', num2str(latency)]);
  pipeline0_1_0_0 : Subsystem  AncestorBlock=casper_library_delays/pipeline  mask(pipeline){latency=fanout_latency}
      mask help:
      | An explicitly laid-out delay line to avoid mapping to SRL16s
      | for use in pipelining to help achieve timing closure.
      mask init:
      | pipeline_init(gcb,'latency',latency);
      settings: AttributesFormatString=Latency = %<latency>
      mask Display:
      | port_label('input', 1, 'd');
      | port_label('output', 1, 'q');
      | disp(['Z^-', num2str(latency)]);
  pipeline0_1_0_1 : Subsystem  AncestorBlock=casper_library_delays/pipeline  mask(pipeline){latency=fanout_latency}
      mask help:
      | An explicitly laid-out delay line to avoid mapping to SRL16s
      | for use in pipelining to help achieve timing closure.
      mask init:
      | pipeline_init(gcb,'latency',latency);
      settings: AttributesFormatString=Latency = %<latency>
      mask Display:
      | port_label('input', 1, 'd');
      | port_label('output', 1, 'q');
      | disp(['Z^-', num2str(latency)]);
  pipeline0_1_0_2 : Subsystem  AncestorBlock=casper_library_delays/pipeline  mask(pipeline){latency=fanout_latency}
      mask help:
      | An explicitly laid-out delay line to avoid mapping to SRL16s
      | for use in pipelining to help achieve timing closure.
      mask init:
      | pipeline_init(gcb,'latency',latency);
      settings: AttributesFormatString=Latency = %<latency>
      mask Display:
      | port_label('input', 1, 'd');
      | port_label('output', 1, 'q');
      | disp(['Z^-', num2str(latency)]);
  pipeline0_1_0_3 : Subsystem  AncestorBlock=casper_library_delays/pipeline  mask(pipeline){latency=fanout_latency}
      mask help:
      | An explicitly laid-out delay line to avoid mapping to SRL16s
      | for use in pipelining to help achieve timing closure.
      mask init:
      | pipeline_init(gcb,'latency',latency);
      settings: AttributesFormatString=Latency = %<latency>
      mask Display:
      | port_label('input', 1, 'd');
      | port_label('output', 1, 'q');
      | disp(['Z^-', num2str(latency)]);
  pipeline0_1_1_0 : Subsystem  AncestorBlock=casper_library_delays/pipeline  mask(pipeline){latency=fanout_latency}
      mask help:
      | An explicitly laid-out delay line to avoid mapping to SRL16s
      | for use in pipelining to help achieve timing closure.
      mask init:
      | pipeline_init(gcb,'latency',latency);
      settings: AttributesFormatString=Latency = %<latency>
      mask Display:
      | port_label('input', 1, 'd');
      | port_label('output', 1, 'q');
      | disp(['Z^-', num2str(latency)]);
  pipeline0_1_1_1 : Subsystem  AncestorBlock=casper_library_delays/pipeline  mask(pipeline){latency=fanout_latency}
      mask help:
      | An explicitly laid-out delay line to avoid mapping to SRL16s
      | for use in pipelining to help achieve timing closure.
      mask init:
      | pipeline_init(gcb,'latency',latency);
      settings: AttributesFormatString=Latency = %<latency>
      mask Display:
      | port_label('input', 1, 'd');
      | port_label('output', 1, 'q');
      | disp(['Z^-', num2str(latency)]);
  pipeline0_1_1_2 : Subsystem  AncestorBlock=casper_library_delays/pipeline  mask(pipeline){latency=fanout_latency}
      mask help:
      | An explicitly laid-out delay line to avoid mapping to SRL16s
      | for use in pipelining to help achieve timing closure.
      mask init:
      | pipeline_init(gcb,'latency',latency);
      settings: AttributesFormatString=Latency = %<latency>
      mask Display:
      | port_label('input', 1, 'd');
      | port_label('output', 1, 'q');
      | disp(['Z^-', num2str(latency)]);
  pipeline0_1_1_3 : Subsystem  AncestorBlock=casper_library_delays/pipeline  mask(pipeline){latency=fanout_latency}
      mask help:
      | An explicitly laid-out delay line to avoid mapping to SRL16s
      | for use in pipelining to help achieve timing closure.
      mask init:
      | pipeline_init(gcb,'latency',latency);
      settings: AttributesFormatString=Latency = %<latency>
      mask Display:
      | port_label('input', 1, 'd');
      | port_label('output', 1, 'q');
      | disp(['Z^-', num2str(latency)]);
  pipeline0_2_0_0 : Subsystem  AncestorBlock=casper_library_delays/pipeline  mask(pipeline){latency=fanout_latency}
      mask help:
      | An explicitly laid-out delay line to avoid mapping to SRL16s
      | for use in pipelining to help achieve timing closure.
      mask init:
      | pipeline_init(gcb,'latency',latency);
      settings: AttributesFormatString=Latency = %<latency>
      mask Display:
      | port_label('input', 1, 'd');
      | port_label('output', 1, 'q');
      | disp(['Z^-', num2str(latency)]);
  pipeline0_2_0_1 : Subsystem  AncestorBlock=casper_library_delays/pipeline  mask(pipeline){latency=fanout_latency}
      mask help:
      | An explicitly laid-out delay line to avoid mapping to SRL16s
      | for use in pipelining to help achieve timing closure.
      mask init:
      | pipeline_init(gcb,'latency',latency);
      settings: AttributesFormatString=Latency = %<latency>
      mask Display:
      | port_label('input', 1, 'd');
      | port_label('output', 1, 'q');
      | disp(['Z^-', num2str(latency)]);
  pipeline0_2_0_2 : Subsystem  AncestorBlock=casper_library_delays/pipeline  mask(pipeline){latency=fanout_latency}
      mask help:
      | An explicitly laid-out delay line to avoid mapping to SRL16s
      | for use in pipelining to help achieve timing closure.
      mask init:
      | pipeline_init(gcb,'latency',latency);
      settings: AttributesFormatString=Latency = %<latency>
      mask Display:
      | port_label('input', 1, 'd');
      | port_label('output', 1, 'q');
      | disp(['Z^-', num2str(latency)]);
  pipeline0_2_0_3 : Subsystem  AncestorBlock=casper_library_delays/pipeline  mask(pipeline){latency=fanout_latency}
      mask help:
      | An explicitly laid-out delay line to avoid mapping to SRL16s
      | for use in pipelining to help achieve timing closure.
      mask init:
      | pipeline_init(gcb,'latency',latency);
      settings: AttributesFormatString=Latency = %<latency>
      mask Display:
      | port_label('input', 1, 'd');
      | port_label('output', 1, 'q');
      | disp(['Z^-', num2str(latency)]);
  pipeline0_2_1_0 : Subsystem  AncestorBlock=casper_library_delays/pipeline  mask(pipeline){latency=fanout_latency}
      mask help:
      | An explicitly laid-out delay line to avoid mapping to SRL16s
      | for use in pipelining to help achieve timing closure.
      mask init:
      | pipeline_init(gcb,'latency',latency);
      settings: AttributesFormatString=Latency = %<latency>
      mask Display:
      | port_label('input', 1, 'd');
      | port_label('output', 1, 'q');
      | disp(['Z^-', num2str(latency)]);
  pipeline0_2_1_1 : Subsystem  AncestorBlock=casper_library_delays/pipeline  mask(pipeline){latency=fanout_latency}
      mask help:
      | An explicitly laid-out delay line to avoid mapping to SRL16s
      | for use in pipelining to help achieve timing closure.
      mask init:
      | pipeline_init(gcb,'latency',latency);
      settings: AttributesFormatString=Latency = %<latency>
      mask Display:
      | port_label('input', 1, 'd');
      | port_label('output', 1, 'q');
      | disp(['Z^-', num2str(latency)]);
  pipeline0_2_1_2 : Subsystem  AncestorBlock=casper_library_delays/pipeline  mask(pipeline){latency=fanout_latency}
      mask help:
      | An explicitly laid-out delay line to avoid mapping to SRL16s
      | for use in pipelining to help achieve timing closure.
      mask init:
      | pipeline_init(gcb,'latency',latency);
      settings: AttributesFormatString=Latency = %<latency>
      mask Display:
      | port_label('input', 1, 'd');
      | port_label('output', 1, 'q');
      | disp(['Z^-', num2str(latency)]);
  pipeline0_2_1_3 : Subsystem  AncestorBlock=casper_library_delays/pipeline  mask(pipeline){latency=fanout_latency}
      mask help:
      | An explicitly laid-out delay line to avoid mapping to SRL16s
      | for use in pipelining to help achieve timing closure.
      mask init:
      | pipeline_init(gcb,'latency',latency);
      settings: AttributesFormatString=Latency = %<latency>
      mask Display:
      | port_label('input', 1, 'd');
      | port_label('output', 1, 'q');
      | disp(['Z^-', num2str(latency)]);
  pipeline0_3_0_0 : Subsystem  AncestorBlock=casper_library_delays/pipeline  mask(pipeline){latency=fanout_latency}
      mask help:
      | An explicitly laid-out delay line to avoid mapping to SRL16s
      | for use in pipelining to help achieve timing closure.
      mask init:
      | pipeline_init(gcb,'latency',latency);
      settings: AttributesFormatString=Latency = %<latency>
      mask Display:
      | port_label('input', 1, 'd');
      | port_label('output', 1, 'q');
      | disp(['Z^-', num2str(latency)]);
  pipeline0_3_0_1 : Subsystem  AncestorBlock=casper_library_delays/pipeline  mask(pipeline){latency=fanout_latency}
      mask help:
      | An explicitly laid-out delay line to avoid mapping to SRL16s
      | for use in pipelining to help achieve timing closure.
      mask init:
      | pipeline_init(gcb,'latency',latency);
      settings: AttributesFormatString=Latency = %<latency>
      mask Display:
      | port_label('input', 1, 'd');
      | port_label('output', 1, 'q');
      | disp(['Z^-', num2str(latency)]);
  pipeline0_3_0_2 : Subsystem  AncestorBlock=casper_library_delays/pipeline  mask(pipeline){latency=fanout_latency}
      mask help:
      | An explicitly laid-out delay line to avoid mapping to SRL16s
      | for use in pipelining to help achieve timing closure.
      mask init:
      | pipeline_init(gcb,'latency',latency);
      settings: AttributesFormatString=Latency = %<latency>
      mask Display:
      | port_label('input', 1, 'd');
      | port_label('output', 1, 'q');
      | disp(['Z^-', num2str(latency)]);
  pipeline0_3_0_3 : Subsystem  AncestorBlock=casper_library_delays/pipeline  mask(pipeline){latency=fanout_latency}
      mask help:
      | An explicitly laid-out delay line to avoid mapping to SRL16s
      | for use in pipelining to help achieve timing closure.
      mask init:
      | pipeline_init(gcb,'latency',latency);
      settings: AttributesFormatString=Latency = %<latency>
      mask Display:
      | port_label('input', 1, 'd');
      | port_label('output', 1, 'q');
      | disp(['Z^-', num2str(latency)]);
  pipeline0_3_1_0 : Subsystem  AncestorBlock=casper_library_delays/pipeline  mask(pipeline){latency=fanout_latency}
      mask help:
      | An explicitly laid-out delay line to avoid mapping to SRL16s
      | for use in pipelining to help achieve timing closure.
      mask init:
      | pipeline_init(gcb,'latency',latency);
      settings: AttributesFormatString=Latency = %<latency>
      mask Display:
      | port_label('input', 1, 'd');
      | port_label('output', 1, 'q');
      | disp(['Z^-', num2str(latency)]);
  pipeline0_3_1_1 : Subsystem  AncestorBlock=casper_library_delays/pipeline  mask(pipeline){latency=fanout_latency}
      mask help:
      | An explicitly laid-out delay line to avoid mapping to SRL16s
      | for use in pipelining to help achieve timing closure.
      mask init:
      | pipeline_init(gcb,'latency',latency);
      settings: AttributesFormatString=Latency = %<latency>
      mask Display:
      | port_label('input', 1, 'd');
      | port_label('output', 1, 'q');
      | disp(['Z^-', num2str(latency)]);
  pipeline0_3_1_2 : Subsystem  AncestorBlock=casper_library_delays/pipeline  mask(pipeline){latency=fanout_latency}
      mask help:
      | An explicitly laid-out delay line to avoid mapping to SRL16s
      | for use in pipelining to help achieve timing closure.
      mask init:
      | pipeline_init(gcb,'latency',latency);
      settings: AttributesFormatString=Latency = %<latency>
      mask Display:
      | port_label('input', 1, 'd');
      | port_label('output', 1, 'q');
      | disp(['Z^-', num2str(latency)]);
  pipeline0_3_1_3 : Subsystem  AncestorBlock=casper_library_delays/pipeline  mask(pipeline){latency=fanout_latency}
      mask help:
      | An explicitly laid-out delay line to avoid mapping to SRL16s
      | for use in pipelining to help achieve timing closure.
      mask init:
      | pipeline_init(gcb,'latency',latency);
      settings: AttributesFormatString=Latency = %<latency>
      mask Display:
      | port_label('input', 1, 'd');
      | port_label('output', 1, 'q');
      | disp(['Z^-', num2str(latency)]);
  pipeline1_0_0_0 : Subsystem  AncestorBlock=casper_library_delays/pipeline  mask(pipeline){latency=fanout_latency}
      mask help:
      | An explicitly laid-out delay line to avoid mapping to SRL16s
      | for use in pipelining to help achieve timing closure.
      mask init:
      | pipeline_init(gcb,'latency',latency);
      settings: AttributesFormatString=Latency = %<latency>
      mask Display:
      | port_label('input', 1, 'd');
      | port_label('output', 1, 'q');
      | disp(['Z^-', num2str(latency)]);
  pipeline1_0_0_1 : Subsystem  AncestorBlock=casper_library_delays/pipeline  mask(pipeline){latency=fanout_latency}
      mask help:
      | An explicitly laid-out delay line to avoid mapping to SRL16s
      | for use in pipelining to help achieve timing closure.
      mask init:
      | pipeline_init(gcb,'latency',latency);
      settings: AttributesFormatString=Latency = %<latency>
      mask Display:
      | port_label('input', 1, 'd');
      | port_label('output', 1, 'q');
      | disp(['Z^-', num2str(latency)]);
  pipeline1_0_0_2 : Subsystem  AncestorBlock=casper_library_delays/pipeline  mask(pipeline){latency=fanout_latency}
      mask help:
      | An explicitly laid-out delay line to avoid mapping to SRL16s
      | for use in pipelining to help achieve timing closure.
      mask init:
      | pipeline_init(gcb,'latency',latency);
      settings: AttributesFormatString=Latency = %<latency>
      mask Display:
      | port_label('input', 1, 'd');
      | port_label('output', 1, 'q');
      | disp(['Z^-', num2str(latency)]);
  pipeline1_0_0_3 : Subsystem  AncestorBlock=casper_library_delays/pipeline  mask(pipeline){latency=fanout_latency}
      mask help:
      | An explicitly laid-out delay line to avoid mapping to SRL16s
      | for use in pipelining to help achieve timing closure.
      mask init:
      | pipeline_init(gcb,'latency',latency);
      settings: AttributesFormatString=Latency = %<latency>
      mask Display:
      | port_label('input', 1, 'd');
      | port_label('output', 1, 'q');
      | disp(['Z^-', num2str(latency)]);
  pipeline1_0_1_0 : Subsystem  AncestorBlock=casper_library_delays/pipeline  mask(pipeline){latency=fanout_latency}
      mask help:
      | An explicitly laid-out delay line to avoid mapping to SRL16s
      | for use in pipelining to help achieve timing closure.
      mask init:
      | pipeline_init(gcb,'latency',latency);
      settings: AttributesFormatString=Latency = %<latency>
      mask Display:
      | port_label('input', 1, 'd');
      | port_label('output', 1, 'q');
      | disp(['Z^-', num2str(latency)]);
  pipeline1_0_1_1 : Subsystem  AncestorBlock=casper_library_delays/pipeline  mask(pipeline){latency=fanout_latency}
      mask help:
      | An explicitly laid-out delay line to avoid mapping to SRL16s
      | for use in pipelining to help achieve timing closure.
      mask init:
      | pipeline_init(gcb,'latency',latency);
      settings: AttributesFormatString=Latency = %<latency>
      mask Display:
      | port_label('input', 1, 'd');
      | port_label('output', 1, 'q');
      | disp(['Z^-', num2str(latency)]);
  pipeline1_0_1_2 : Subsystem  AncestorBlock=casper_library_delays/pipeline  mask(pipeline){latency=fanout_latency}
      mask help:
      | An explicitly laid-out delay line to avoid mapping to SRL16s
      | for use in pipelining to help achieve timing closure.
      mask init:
      | pipeline_init(gcb,'latency',latency);
      settings: AttributesFormatString=Latency = %<latency>
      mask Display:
      | port_label('input', 1, 'd');
      | port_label('output', 1, 'q');
      | disp(['Z^-', num2str(latency)]);
  pipeline1_0_1_3 : Subsystem  AncestorBlock=casper_library_delays/pipeline  mask(pipeline){latency=fanout_latency}
      mask help:
      | An explicitly laid-out delay line to avoid mapping to SRL16s
      | for use in pipelining to help achieve timing closure.
      mask init:
      | pipeline_init(gcb,'latency',latency);
      settings: AttributesFormatString=Latency = %<latency>
      mask Display:
      | port_label('input', 1, 'd');
      | port_label('output', 1, 'q');
      | disp(['Z^-', num2str(latency)]);
  pipeline1_1_0_0 : Subsystem  AncestorBlock=casper_library_delays/pipeline  mask(pipeline){latency=fanout_latency}
      mask help:
      | An explicitly laid-out delay line to avoid mapping to SRL16s
      | for use in pipelining to help achieve timing closure.
      mask init:
      | pipeline_init(gcb,'latency',latency);
      settings: AttributesFormatString=Latency = %<latency>
      mask Display:
      | port_label('input', 1, 'd');
      | port_label('output', 1, 'q');
      | disp(['Z^-', num2str(latency)]);
  pipeline1_1_0_1 : Subsystem  AncestorBlock=casper_library_delays/pipeline  mask(pipeline){latency=fanout_latency}
      mask help:
      | An explicitly laid-out delay line to avoid mapping to SRL16s
      | for use in pipelining to help achieve timing closure.
      mask init:
      | pipeline_init(gcb,'latency',latency);
      settings: AttributesFormatString=Latency = %<latency>
      mask Display:
      | port_label('input', 1, 'd');
      | port_label('output', 1, 'q');
      | disp(['Z^-', num2str(latency)]);
  pipeline1_1_0_2 : Subsystem  AncestorBlock=casper_library_delays/pipeline  mask(pipeline){latency=fanout_latency}
      mask help:
      | An explicitly laid-out delay line to avoid mapping to SRL16s
      | for use in pipelining to help achieve timing closure.
      mask init:
      | pipeline_init(gcb,'latency',latency);
      settings: AttributesFormatString=Latency = %<latency>
      mask Display:
      | port_label('input', 1, 'd');
      | port_label('output', 1, 'q');
      | disp(['Z^-', num2str(latency)]);
  pipeline1_1_0_3 : Subsystem  AncestorBlock=casper_library_delays/pipeline  mask(pipeline){latency=fanout_latency}
      mask help:
      | An explicitly laid-out delay line to avoid mapping to SRL16s
      | for use in pipelining to help achieve timing closure.
      mask init:
      | pipeline_init(gcb,'latency',latency);
      settings: AttributesFormatString=Latency = %<latency>
      mask Display:
      | port_label('input', 1, 'd');
      | port_label('output', 1, 'q');
      | disp(['Z^-', num2str(latency)]);
  pipeline1_1_1_0 : Subsystem  AncestorBlock=casper_library_delays/pipeline  mask(pipeline){latency=fanout_latency}
      mask help:
      | An explicitly laid-out delay line to avoid mapping to SRL16s
      | for use in pipelining to help achieve timing closure.
      mask init:
      | pipeline_init(gcb,'latency',latency);
      settings: AttributesFormatString=Latency = %<latency>
      mask Display:
      | port_label('input', 1, 'd');
      | port_label('output', 1, 'q');
      | disp(['Z^-', num2str(latency)]);
  pipeline1_1_1_1 : Subsystem  AncestorBlock=casper_library_delays/pipeline  mask(pipeline){latency=fanout_latency}
      mask help:
      | An explicitly laid-out delay line to avoid mapping to SRL16s
      | for use in pipelining to help achieve timing closure.
      mask init:
      | pipeline_init(gcb,'latency',latency);
      settings: AttributesFormatString=Latency = %<latency>
      mask Display:
      | port_label('input', 1, 'd');
      | port_label('output', 1, 'q');
      | disp(['Z^-', num2str(latency)]);
  pipeline1_1_1_2 : Subsystem  AncestorBlock=casper_library_delays/pipeline  mask(pipeline){latency=fanout_latency}
      mask help:
      | An explicitly laid-out delay line to avoid mapping to SRL16s
      | for use in pipelining to help achieve timing closure.
      mask init:
      | pipeline_init(gcb,'latency',latency);
      settings: AttributesFormatString=Latency = %<latency>
      mask Display:
      | port_label('input', 1, 'd');
      | port_label('output', 1, 'q');
      | disp(['Z^-', num2str(latency)]);
  pipeline1_1_1_3 : Subsystem  AncestorBlock=casper_library_delays/pipeline  mask(pipeline){latency=fanout_latency}
      mask help:
      | An explicitly laid-out delay line to avoid mapping to SRL16s
      | for use in pipelining to help achieve timing closure.
      mask init:
      | pipeline_init(gcb,'latency',latency);
      settings: AttributesFormatString=Latency = %<latency>
      mask Display:
      | port_label('input', 1, 'd');
      | port_label('output', 1, 'q');
      | disp(['Z^-', num2str(latency)]);
  pipeline1_2_0_0 : Subsystem  AncestorBlock=casper_library_delays/pipeline  mask(pipeline){latency=fanout_latency}
      mask help:
      | An explicitly laid-out delay line to avoid mapping to SRL16s
      | for use in pipelining to help achieve timing closure.
      mask init:
      | pipeline_init(gcb,'latency',latency);
      settings: AttributesFormatString=Latency = %<latency>
      mask Display:
      | port_label('input', 1, 'd');
      | port_label('output', 1, 'q');
      | disp(['Z^-', num2str(latency)]);
  pipeline1_2_0_1 : Subsystem  AncestorBlock=casper_library_delays/pipeline  mask(pipeline){latency=fanout_latency}
      mask help:
      | An explicitly laid-out delay line to avoid mapping to SRL16s
      | for use in pipelining to help achieve timing closure.
      mask init:
      | pipeline_init(gcb,'latency',latency);
      settings: AttributesFormatString=Latency = %<latency>
      mask Display:
      | port_label('input', 1, 'd');
      | port_label('output', 1, 'q');
      | disp(['Z^-', num2str(latency)]);
  pipeline1_2_0_2 : Subsystem  AncestorBlock=casper_library_delays/pipeline  mask(pipeline){latency=fanout_latency}
      mask help:
      | An explicitly laid-out delay line to avoid mapping to SRL16s
      | for use in pipelining to help achieve timing closure.
      mask init:
      | pipeline_init(gcb,'latency',latency);
      settings: AttributesFormatString=Latency = %<latency>
      mask Display:
      | port_label('input', 1, 'd');
      | port_label('output', 1, 'q');
      | disp(['Z^-', num2str(latency)]);
  pipeline1_2_0_3 : Subsystem  AncestorBlock=casper_library_delays/pipeline  mask(pipeline){latency=fanout_latency}
      mask help:
      | An explicitly laid-out delay line to avoid mapping to SRL16s
      | for use in pipelining to help achieve timing closure.
      mask init:
      | pipeline_init(gcb,'latency',latency);
      settings: AttributesFormatString=Latency = %<latency>
      mask Display:
      | port_label('input', 1, 'd');
      | port_label('output', 1, 'q');
      | disp(['Z^-', num2str(latency)]);
  pipeline1_2_1_0 : Subsystem  AncestorBlock=casper_library_delays/pipeline  mask(pipeline){latency=fanout_latency}
      mask help:
      | An explicitly laid-out delay line to avoid mapping to SRL16s
      | for use in pipelining to help achieve timing closure.
      mask init:
      | pipeline_init(gcb,'latency',latency);
      settings: AttributesFormatString=Latency = %<latency>
      mask Display:
      | port_label('input', 1, 'd');
      | port_label('output', 1, 'q');
      | disp(['Z^-', num2str(latency)]);
  pipeline1_2_1_1 : Subsystem  AncestorBlock=casper_library_delays/pipeline  mask(pipeline){latency=fanout_latency}
      mask help:
      | An explicitly laid-out delay line to avoid mapping to SRL16s
      | for use in pipelining to help achieve timing closure.
      mask init:
      | pipeline_init(gcb,'latency',latency);
      settings: AttributesFormatString=Latency = %<latency>
      mask Display:
      | port_label('input', 1, 'd');
      | port_label('output', 1, 'q');
      | disp(['Z^-', num2str(latency)]);
  pipeline1_2_1_2 : Subsystem  AncestorBlock=casper_library_delays/pipeline  mask(pipeline){latency=fanout_latency}
      mask help:
      | An explicitly laid-out delay line to avoid mapping to SRL16s
      | for use in pipelining to help achieve timing closure.
      mask init:
      | pipeline_init(gcb,'latency',latency);
      settings: AttributesFormatString=Latency = %<latency>
      mask Display:
      | port_label('input', 1, 'd');
      | port_label('output', 1, 'q');
      | disp(['Z^-', num2str(latency)]);
  pipeline1_2_1_3 : Subsystem  AncestorBlock=casper_library_delays/pipeline  mask(pipeline){latency=fanout_latency}
      mask help:
      | An explicitly laid-out delay line to avoid mapping to SRL16s
      | for use in pipelining to help achieve timing closure.
      mask init:
      | pipeline_init(gcb,'latency',latency);
      settings: AttributesFormatString=Latency = %<latency>
      mask Display:
      | port_label('input', 1, 'd');
      | port_label('output', 1, 'q');
      | disp(['Z^-', num2str(latency)]);
  pipeline2_0_0_0 : Subsystem  AncestorBlock=casper_library_delays/pipeline  mask(pipeline){latency=fanout_latency}
      mask help:
      | An explicitly laid-out delay line to avoid mapping to SRL16s
      | for use in pipelining to help achieve timing closure.
      mask init:
      | pipeline_init(gcb,'latency',latency);
      settings: AttributesFormatString=Latency = %<latency>
      mask Display:
      | port_label('input', 1, 'd');
      | port_label('output', 1, 'q');
      | disp(['Z^-', num2str(latency)]);
  pipeline2_0_0_1 : Subsystem  AncestorBlock=casper_library_delays/pipeline  mask(pipeline){latency=fanout_latency}
      mask help:
      | An explicitly laid-out delay line to avoid mapping to SRL16s
      | for use in pipelining to help achieve timing closure.
      mask init:
      | pipeline_init(gcb,'latency',latency);
      settings: AttributesFormatString=Latency = %<latency>
      mask Display:
      | port_label('input', 1, 'd');
      | port_label('output', 1, 'q');
      | disp(['Z^-', num2str(latency)]);
  pipeline2_0_0_2 : Subsystem  AncestorBlock=casper_library_delays/pipeline  mask(pipeline){latency=fanout_latency}
      mask help:
      | An explicitly laid-out delay line to avoid mapping to SRL16s
      | for use in pipelining to help achieve timing closure.
      mask init:
      | pipeline_init(gcb,'latency',latency);
      settings: AttributesFormatString=Latency = %<latency>
      mask Display:
      | port_label('input', 1, 'd');
      | port_label('output', 1, 'q');
      | disp(['Z^-', num2str(latency)]);
  pipeline2_0_0_3 : Subsystem  AncestorBlock=casper_library_delays/pipeline  mask(pipeline){latency=fanout_latency}
      mask help:
      | An explicitly laid-out delay line to avoid mapping to SRL16s
      | for use in pipelining to help achieve timing closure.
      mask init:
      | pipeline_init(gcb,'latency',latency);
      settings: AttributesFormatString=Latency = %<latency>
      mask Display:
      | port_label('input', 1, 'd');
      | port_label('output', 1, 'q');
      | disp(['Z^-', num2str(latency)]);
  pipeline2_0_1_0 : Subsystem  AncestorBlock=casper_library_delays/pipeline  mask(pipeline){latency=fanout_latency}
      mask help:
      | An explicitly laid-out delay line to avoid mapping to SRL16s
      | for use in pipelining to help achieve timing closure.
      mask init:
      | pipeline_init(gcb,'latency',latency);
      settings: AttributesFormatString=Latency = %<latency>
      mask Display:
      | port_label('input', 1, 'd');
      | port_label('output', 1, 'q');
      | disp(['Z^-', num2str(latency)]);
  pipeline2_0_1_1 : Subsystem  AncestorBlock=casper_library_delays/pipeline  mask(pipeline){latency=fanout_latency}
      mask help:
      | An explicitly laid-out delay line to avoid mapping to SRL16s
      | for use in pipelining to help achieve timing closure.
      mask init:
      | pipeline_init(gcb,'latency',latency);
      settings: AttributesFormatString=Latency = %<latency>
      mask Display:
      | port_label('input', 1, 'd');
      | port_label('output', 1, 'q');
      | disp(['Z^-', num2str(latency)]);
  pipeline2_0_1_2 : Subsystem  AncestorBlock=casper_library_delays/pipeline  mask(pipeline){latency=fanout_latency}
      mask help:
      | An explicitly laid-out delay line to avoid mapping to SRL16s
      | for use in pipelining to help achieve timing closure.
      mask init:
      | pipeline_init(gcb,'latency',latency);
      settings: AttributesFormatString=Latency = %<latency>
      mask Display:
      | port_label('input', 1, 'd');
      | port_label('output', 1, 'q');
      | disp(['Z^-', num2str(latency)]);
  pipeline2_0_1_3 : Subsystem  AncestorBlock=casper_library_delays/pipeline  mask(pipeline){latency=fanout_latency}
      mask help:
      | An explicitly laid-out delay line to avoid mapping to SRL16s
      | for use in pipelining to help achieve timing closure.
      mask init:
      | pipeline_init(gcb,'latency',latency);
      settings: AttributesFormatString=Latency = %<latency>
      mask Display:
      | port_label('input', 1, 'd');
      | port_label('output', 1, 'q');
      | disp(['Z^-', num2str(latency)]);
  pipeline2_1_0_0 : Subsystem  AncestorBlock=casper_library_delays/pipeline  mask(pipeline){latency=fanout_latency}
      mask help:
      | An explicitly laid-out delay line to avoid mapping to SRL16s
      | for use in pipelining to help achieve timing closure.
      mask init:
      | pipeline_init(gcb,'latency',latency);
      settings: AttributesFormatString=Latency = %<latency>
      mask Display:
      | port_label('input', 1, 'd');
      | port_label('output', 1, 'q');
      | disp(['Z^-', num2str(latency)]);
  pipeline2_1_0_1 : Subsystem  AncestorBlock=casper_library_delays/pipeline  mask(pipeline){latency=fanout_latency}
      mask help:
      | An explicitly laid-out delay line to avoid mapping to SRL16s
      | for use in pipelining to help achieve timing closure.
      mask init:
      | pipeline_init(gcb,'latency',latency);
      settings: AttributesFormatString=Latency = %<latency>
      mask Display:
      | port_label('input', 1, 'd');
      | port_label('output', 1, 'q');
      | disp(['Z^-', num2str(latency)]);
  pipeline2_1_0_2 : Subsystem  AncestorBlock=casper_library_delays/pipeline  mask(pipeline){latency=fanout_latency}
      mask help:
      | An explicitly laid-out delay line to avoid mapping to SRL16s
      | for use in pipelining to help achieve timing closure.
      mask init:
      | pipeline_init(gcb,'latency',latency);
      settings: AttributesFormatString=Latency = %<latency>
      mask Display:
      | port_label('input', 1, 'd');
      | port_label('output', 1, 'q');
      | disp(['Z^-', num2str(latency)]);
  pipeline2_1_0_3 : Subsystem  AncestorBlock=casper_library_delays/pipeline  mask(pipeline){latency=fanout_latency}
      mask help:
      | An explicitly laid-out delay line to avoid mapping to SRL16s
      | for use in pipelining to help achieve timing closure.
      mask init:
      | pipeline_init(gcb,'latency',latency);
      settings: AttributesFormatString=Latency = %<latency>
      mask Display:
      | port_label('input', 1, 'd');
      | port_label('output', 1, 'q');
      | disp(['Z^-', num2str(latency)]);
  pipeline2_1_1_0 : Subsystem  AncestorBlock=casper_library_delays/pipeline  mask(pipeline){latency=fanout_latency}
      mask help:
      | An explicitly laid-out delay line to avoid mapping to SRL16s
      | for use in pipelining to help achieve timing closure.
      mask init:
      | pipeline_init(gcb,'latency',latency);
      settings: AttributesFormatString=Latency = %<latency>
      mask Display:
      | port_label('input', 1, 'd');
      | port_label('output', 1, 'q');
      | disp(['Z^-', num2str(latency)]);
  pipeline2_1_1_1 : Subsystem  AncestorBlock=casper_library_delays/pipeline  mask(pipeline){latency=fanout_latency}
      mask help:
      | An explicitly laid-out delay line to avoid mapping to SRL16s
      | for use in pipelining to help achieve timing closure.
      mask init:
      | pipeline_init(gcb,'latency',latency);
      settings: AttributesFormatString=Latency = %<latency>
      mask Display:
      | port_label('input', 1, 'd');
      | port_label('output', 1, 'q');
      | disp(['Z^-', num2str(latency)]);
  pipeline2_1_1_2 : Subsystem  AncestorBlock=casper_library_delays/pipeline  mask(pipeline){latency=fanout_latency}
      mask help:
      | An explicitly laid-out delay line to avoid mapping to SRL16s
      | for use in pipelining to help achieve timing closure.
      mask init:
      | pipeline_init(gcb,'latency',latency);
      settings: AttributesFormatString=Latency = %<latency>
      mask Display:
      | port_label('input', 1, 'd');
      | port_label('output', 1, 'q');
      | disp(['Z^-', num2str(latency)]);
  pipeline2_1_1_3 : Subsystem  AncestorBlock=casper_library_delays/pipeline  mask(pipeline){latency=fanout_latency}
      mask help:
      | An explicitly laid-out delay line to avoid mapping to SRL16s
      | for use in pipelining to help achieve timing closure.
      mask init:
      | pipeline_init(gcb,'latency',latency);
      settings: AttributesFormatString=Latency = %<latency>
      mask Display:
      | port_label('input', 1, 'd');
      | port_label('output', 1, 'q');
      | disp(['Z^-', num2str(latency)]);
  pipeline3_0_0_0 : Subsystem  AncestorBlock=casper_library_delays/pipeline  mask(pipeline){latency=fanout_latency}
      mask help:
      | An explicitly laid-out delay line to avoid mapping to SRL16s
      | for use in pipelining to help achieve timing closure.
      mask init:
      | pipeline_init(gcb,'latency',latency);
      settings: AttributesFormatString=Latency = %<latency>
      mask Display:
      | port_label('input', 1, 'd');
      | port_label('output', 1, 'q');
      | disp(['Z^-', num2str(latency)]);
  pipeline3_0_0_1 : Subsystem  AncestorBlock=casper_library_delays/pipeline  mask(pipeline){latency=fanout_latency}
      mask help:
      | An explicitly laid-out delay line to avoid mapping to SRL16s
      | for use in pipelining to help achieve timing closure.
      mask init:
      | pipeline_init(gcb,'latency',latency);
      settings: AttributesFormatString=Latency = %<latency>
      mask Display:
      | port_label('input', 1, 'd');
      | port_label('output', 1, 'q');
      | disp(['Z^-', num2str(latency)]);
  pipeline3_0_0_2 : Subsystem  AncestorBlock=casper_library_delays/pipeline  mask(pipeline){latency=fanout_latency}
      mask help:
      | An explicitly laid-out delay line to avoid mapping to SRL16s
      | for use in pipelining to help achieve timing closure.
      mask init:
      | pipeline_init(gcb,'latency',latency);
      settings: AttributesFormatString=Latency = %<latency>
      mask Display:
      | port_label('input', 1, 'd');
      | port_label('output', 1, 'q');
      | disp(['Z^-', num2str(latency)]);
  pipeline3_0_0_3 : Subsystem  AncestorBlock=casper_library_delays/pipeline  mask(pipeline){latency=fanout_latency}
      mask help:
      | An explicitly laid-out delay line to avoid mapping to SRL16s
      | for use in pipelining to help achieve timing closure.
      mask init:
      | pipeline_init(gcb,'latency',latency);
      settings: AttributesFormatString=Latency = %<latency>
      mask Display:
      | port_label('input', 1, 'd');
      | port_label('output', 1, 'q');
      | disp(['Z^-', num2str(latency)]);
  pipeline3_0_1_0 : Subsystem  AncestorBlock=casper_library_delays/pipeline  mask(pipeline){latency=fanout_latency}
      mask help:
      | An explicitly laid-out delay line to avoid mapping to SRL16s
      | for use in pipelining to help achieve timing closure.
      mask init:
      | pipeline_init(gcb,'latency',latency);
      settings: AttributesFormatString=Latency = %<latency>
      mask Display:
      | port_label('input', 1, 'd');
      | port_label('output', 1, 'q');
      | disp(['Z^-', num2str(latency)]);
  pipeline3_0_1_1 : Subsystem  AncestorBlock=casper_library_delays/pipeline  mask(pipeline){latency=fanout_latency}
      mask help:
      | An explicitly laid-out delay line to avoid mapping to SRL16s
      | for use in pipelining to help achieve timing closure.
      mask init:
      | pipeline_init(gcb,'latency',latency);
      settings: AttributesFormatString=Latency = %<latency>
      mask Display:
      | port_label('input', 1, 'd');
      | port_label('output', 1, 'q');
      | disp(['Z^-', num2str(latency)]);
  pipeline3_0_1_2 : Subsystem  AncestorBlock=casper_library_delays/pipeline  mask(pipeline){latency=fanout_latency}
      mask help:
      | An explicitly laid-out delay line to avoid mapping to SRL16s
      | for use in pipelining to help achieve timing closure.
      mask init:
      | pipeline_init(gcb,'latency',latency);
      settings: AttributesFormatString=Latency = %<latency>
      mask Display:
      | port_label('input', 1, 'd');
      | port_label('output', 1, 'q');
      | disp(['Z^-', num2str(latency)]);
  pipeline3_0_1_3 : Subsystem  AncestorBlock=casper_library_delays/pipeline  mask(pipeline){latency=fanout_latency}
      mask help:
      | An explicitly laid-out delay line to avoid mapping to SRL16s
      | for use in pipelining to help achieve timing closure.
      mask init:
      | pipeline_init(gcb,'latency',latency);
      settings: AttributesFormatString=Latency = %<latency>
      mask Display:
      | port_label('input', 1, 'd');
      | port_label('output', 1, 'q');
      | disp(['Z^-', num2str(latency)]);
  ri_to_c0_0_0 : casper_library_misc/ri_to_c
  ri_to_c0_0_1 : casper_library_misc/ri_to_c
  ri_to_c0_1_0 : casper_library_misc/ri_to_c
  ri_to_c0_1_1 : casper_library_misc/ri_to_c
  ri_to_c0_2_0 : casper_library_misc/ri_to_c
  ri_to_c0_2_1 : casper_library_misc/ri_to_c
  ri_to_c0_3_0 : casper_library_misc/ri_to_c
  ri_to_c0_3_1 : casper_library_misc/ri_to_c
  ri_to_c1_0_0 : casper_library_misc/ri_to_c
  ri_to_c1_0_1 : casper_library_misc/ri_to_c
  ri_to_c1_1_0 : casper_library_misc/ri_to_c
  ri_to_c1_1_1 : casper_library_misc/ri_to_c
  ri_to_c1_2_0 : casper_library_misc/ri_to_c
  ri_to_c1_2_1 : casper_library_misc/ri_to_c
  ri_to_c2_0_0 : casper_library_misc/ri_to_c
  ri_to_c2_0_1 : casper_library_misc/ri_to_c
  ri_to_c2_1_0 : casper_library_misc/ri_to_c
  ri_to_c2_1_1 : casper_library_misc/ri_to_c
  ri_to_c3_0_0 : casper_library_misc/ri_to_c
  ri_to_c3_0_1 : casper_library_misc/ri_to_c
  sync_delay : xbsIndex_r4/Delay  rst=off  infoeditControl=Selection of Reset will increase slice count due to use of real FFs and instead of SRLs  en=off  latency=mult_latency+add_latency+conv_latency+fanout_latency  dbl_ovrd=off  reg_retiming=off  block_type=delay
  unpack0 : Subsystem  AncestorBlock=casper_library_flow_control/bus_expand  mask(bus_expand){mode=divisions of equal size, outputNum=aggregation, outputWidth=bit_width_in*2, outputBinaryPt=0, outputArithmeticType=0, show_format=off, outputToWorkspace=off, variablePrefix=out, outputToModelAsWell=on}
      mask prompts: outputNum "Number of outputs:"; outputWidth "Output width:"; outputBinaryPt "Output binary point position:"; outputArithmeticType "Output arithmetic type (ufix=0, fix=1, bool=2):"; show_format "Print format string?"; outputToWorkspace "Output to workspace?"; variablePrefix "Variable name prefix:"; outputToModelAsWell "Output to model as well?"
      mask help:
      | Expands a 'bus' made using a bus_create or Xilinx
      | concat block.
      | The input will be divided into the specified number
      | of outputs with the specified arithmetic types.
      | Divisions are made from most significant bit.
      mask init: same as fft_4ch_nofir/bus_expand
      settings: AttributesFormatString=2 outputs
      mask TypeOptions mode: divisions of equal size | divisions of arbitrary size
      mask Callback mode: bus_expand_callback();
      mask Callback outputWidth: bus_expand_callback();
      mask Callback outputToWorkspace: bus_expand_callback();
  unpack1 : Subsystem  AncestorBlock=casper_library_flow_control/bus_expand  mask(bus_expand){mode=divisions of equal size, outputNum=aggregation, outputWidth=bit_width_in*2, outputBinaryPt=0, outputArithmeticType=0, show_format=off, outputToWorkspace=off, variablePrefix=out, outputToModelAsWell=on}
      mask prompts: outputNum "Number of outputs:"; outputWidth "Output width:"; outputBinaryPt "Output binary point position:"; outputArithmeticType "Output arithmetic type (ufix=0, fix=1, bool=2):"; show_format "Print format string?"; outputToWorkspace "Output to workspace?"; variablePrefix "Variable name prefix:"; outputToModelAsWell "Output to model as well?"
      mask help:
      | Expands a 'bus' made using a bus_create or Xilinx
      | concat block.
      | The input will be divided into the specified number
      | of outputs with the specified arithmetic types.
      | Divisions are made from most significant bit.
      mask init: same as fft_4ch_nofir/bus_expand
      settings: AttributesFormatString=2 outputs
      mask TypeOptions mode: divisions of equal size | divisions of arbitrary size
      mask Callback mode: bus_expand_callback();
      mask Callback outputWidth: bus_expand_callback();
      mask Callback outputToWorkspace: bus_expand_callback();
  unpack2 : Subsystem  AncestorBlock=casper_library_flow_control/bus_expand  mask(bus_expand){mode=divisions of equal size, outputNum=aggregation, outputWidth=bit_width_in*2, outputBinaryPt=0, outputArithmeticType=0, show_format=off, outputToWorkspace=off, variablePrefix=out, outputToModelAsWell=on}
      mask prompts: outputNum "Number of outputs:"; outputWidth "Output width:"; outputBinaryPt "Output binary point position:"; outputArithmeticType "Output arithmetic type (ufix=0, fix=1, bool=2):"; show_format "Print format string?"; outputToWorkspace "Output to workspace?"; variablePrefix "Variable name prefix:"; outputToModelAsWell "Output to model as well?"
      mask help:
      | Expands a 'bus' made using a bus_create or Xilinx
      | concat block.
      | The input will be divided into the specified number
      | of outputs with the specified arithmetic types.
      | Divisions are made from most significant bit.
      mask init: same as fft_4ch_nofir/bus_expand
      settings: AttributesFormatString=2 outputs
      mask TypeOptions mode: divisions of equal size | divisions of arbitrary size
      mask Callback mode: bus_expand_callback();
      mask Callback outputWidth: bus_expand_callback();
      mask Callback outputToWorkspace: bus_expand_callback();
  unpack3 : Subsystem  AncestorBlock=casper_library_flow_control/bus_expand  mask(bus_expand){mode=divisions of equal size, outputNum=aggregation, outputWidth=bit_width_in*2, outputBinaryPt=0, outputArithmeticType=0, show_format=off, outputToWorkspace=off, variablePrefix=out, outputToModelAsWell=on}
      mask prompts: outputNum "Number of outputs:"; outputWidth "Output width:"; outputBinaryPt "Output binary point position:"; outputArithmeticType "Output arithmetic type (ufix=0, fix=1, bool=2):"; show_format "Print format string?"; outputToWorkspace "Output to workspace?"; variablePrefix "Variable name prefix:"; outputToModelAsWell "Output to model as well?"
      mask help:
      | Expands a 'bus' made using a bus_create or Xilinx
      | concat block.
      | The input will be divided into the specified number
      | of outputs with the specified arithmetic types.
      | Divisions are made from most significant bit.
      mask init: same as fft_4ch_nofir/bus_expand
      settings: AttributesFormatString=2 outputs
      mask TypeOptions mode: divisions of equal size | divisions of arbitrary size
      mask Callback mode: bus_expand_callback();
      mask Callback outputWidth: bus_expand_callback();
      mask Callback outputToWorkspace: bus_expand_callback();
  sync_out : Outport
  din0_x_din0* : Outport  Port=2
  din0_x_din1* : Outport  Port=3
  din0_x_din2* : Outport  Port=4
  din0_x_din3* : Outport  Port=5
  din1_x_din1* : Outport  Port=6
  din1_x_din2* : Outport  Port=7
  din1_x_din3* : Outport  Port=8
  din2_x_din2* : Outport  Port=9
  din2_x_din3* : Outport  Port=10
  din3_x_din3* : Outport  Port=11
  wires:
  sync_in/1 -> sync_delay/1
  sync_delay/1 -> sync_out/1
  din0/1 -> unpack0/1(bus_in)
  unpack0/1(msb_out2) -> c_to_ri0_0/1
  unpack0/2(lsb_out1) -> c_to_ri0_1/1
  din1/1 -> unpack1/1(bus_in)
  unpack1/1(msb_out2) -> c_to_ri1_0/1
  unpack1/2(lsb_out1) -> c_to_ri1_1/1
  din2/1 -> unpack2/1(bus_in)
  unpack2/1(msb_out2) -> c_to_ri2_0/1
  unpack2/2(lsb_out1) -> c_to_ri2_1/1
  din3/1 -> unpack3/1(bus_in)
  unpack3/1(msb_out2) -> c_to_ri3_0/1
  unpack3/2(lsb_out1) -> c_to_ri3_1/1
  c_to_ri0_0/1 -> pipeline0_0_0_0/1(d), pipeline0_0_0_2/1(d), pipeline0_1_0_0/1(d), pipeline0_2_0_0/1(d), pipeline0_3_0_0/1(d)
  pipeline0_0_0_0/1(q) -> cmult0_0_0/1
  c_to_ri0_0/2 -> pipeline0_0_0_1/1(d), pipeline0_0_0_3/1(d), pipeline0_1_0_1/1(d), pipeline0_2_0_1/1(d), pipeline0_3_0_1/1(d)
  pipeline0_0_0_1/1(q) -> cmult0_0_0/2
  pipeline0_0_0_2/1(q) -> cmult0_0_0/3
  pipeline0_0_0_3/1(q) -> cmult0_0_0/4
  cmult0_0_0/1 -> cvrt0_0_0_real/1(din)
  cmult0_0_0/2 -> cvrt0_0_0_imag/1(din)
  cvrt0_0_0_real/1(dout) -> ri_to_c0_0_0/1
  cvrt0_0_0_imag/1(dout) -> ri_to_c0_0_0/2
  ri_to_c0_0_0/1 -> pack0_0/1(in1)
  c_to_ri0_1/1 -> pipeline0_0_1_0/1(d), pipeline0_0_1_2/1(d), pipeline0_1_1_0/1(d), pipeline0_2_1_0/1(d), pipeline0_3_1_0/1(d)
  pipeline0_0_1_0/1(q) -> cmult0_0_1/1
  c_to_ri0_1/2 -> pipeline0_0_1_1/1(d), pipeline0_0_1_3/1(d), pipeline0_1_1_1/1(d), pipeline0_2_1_1/1(d), pipeline0_3_1_1/1(d)
  pipeline0_0_1_1/1(q) -> cmult0_0_1/2
  pipeline0_0_1_2/1(q) -> cmult0_0_1/3
  pipeline0_0_1_3/1(q) -> cmult0_0_1/4
  cmult0_0_1/1 -> cvrt0_0_1_real/1(din)
  cmult0_0_1/2 -> cvrt0_0_1_imag/1(din)
  cvrt0_0_1_real/1(dout) -> ri_to_c0_0_1/1
  cvrt0_0_1_imag/1(dout) -> ri_to_c0_0_1/2
  ri_to_c0_0_1/1 -> pack0_0/2(in2)
  pack0_0/1(bus_out) -> din0_x_din0*/1
  pipeline0_1_0_0/1(q) -> cmult0_1_0/1
  pipeline0_1_0_1/1(q) -> cmult0_1_0/2
  c_to_ri1_0/1 -> pipeline0_1_0_2/1(d), pipeline1_0_0_0/1(d), pipeline1_0_0_2/1(d), pipeline1_1_0_0/1(d), pipeline1_2_0_0/1(d)
  pipeline0_1_0_2/1(q) -> cmult0_1_0/3
  c_to_ri1_0/2 -> pipeline0_1_0_3/1(d), pipeline1_0_0_1/1(d), pipeline1_0_0_3/1(d), pipeline1_1_0_1/1(d), pipeline1_2_0_1/1(d)
  pipeline0_1_0_3/1(q) -> cmult0_1_0/4
  cmult0_1_0/1 -> cvrt0_1_0_real/1(din)
  cmult0_1_0/2 -> cvrt0_1_0_imag/1(din)
  cvrt0_1_0_real/1(dout) -> ri_to_c0_1_0/1
  cvrt0_1_0_imag/1(dout) -> ri_to_c0_1_0/2
  ri_to_c0_1_0/1 -> pack0_1/1(in1)
  pipeline0_1_1_0/1(q) -> cmult0_1_1/1
  pipeline0_1_1_1/1(q) -> cmult0_1_1/2
  c_to_ri1_1/1 -> pipeline0_1_1_2/1(d), pipeline1_0_1_0/1(d), pipeline1_0_1_2/1(d), pipeline1_1_1_0/1(d), pipeline1_2_1_0/1(d)
  pipeline0_1_1_2/1(q) -> cmult0_1_1/3
  c_to_ri1_1/2 -> pipeline0_1_1_3/1(d), pipeline1_0_1_1/1(d), pipeline1_0_1_3/1(d), pipeline1_1_1_1/1(d), pipeline1_2_1_1/1(d)
  pipeline0_1_1_3/1(q) -> cmult0_1_1/4
  cmult0_1_1/1 -> cvrt0_1_1_real/1(din)
  cmult0_1_1/2 -> cvrt0_1_1_imag/1(din)
  cvrt0_1_1_real/1(dout) -> ri_to_c0_1_1/1
  cvrt0_1_1_imag/1(dout) -> ri_to_c0_1_1/2
  ri_to_c0_1_1/1 -> pack0_1/2(in2)
  pack0_1/1(bus_out) -> din0_x_din1*/1
  pipeline0_2_0_0/1(q) -> cmult0_2_0/1
  pipeline0_2_0_1/1(q) -> cmult0_2_0/2
  c_to_ri2_0/1 -> pipeline0_2_0_2/1(d), pipeline1_1_0_2/1(d), pipeline2_0_0_0/1(d), pipeline2_0_0_2/1(d), pipeline2_1_0_0/1(d)
  pipeline0_2_0_2/1(q) -> cmult0_2_0/3
  c_to_ri2_0/2 -> pipeline0_2_0_3/1(d), pipeline1_1_0_3/1(d), pipeline2_0_0_1/1(d), pipeline2_0_0_3/1(d), pipeline2_1_0_1/1(d)
  pipeline0_2_0_3/1(q) -> cmult0_2_0/4
  cmult0_2_0/1 -> cvrt0_2_0_real/1(din)
  cmult0_2_0/2 -> cvrt0_2_0_imag/1(din)
  cvrt0_2_0_real/1(dout) -> ri_to_c0_2_0/1
  cvrt0_2_0_imag/1(dout) -> ri_to_c0_2_0/2
  ri_to_c0_2_0/1 -> pack0_2/1(in1)
  pipeline0_2_1_0/1(q) -> cmult0_2_1/1
  pipeline0_2_1_1/1(q) -> cmult0_2_1/2
  c_to_ri2_1/1 -> pipeline0_2_1_2/1(d), pipeline1_1_1_2/1(d), pipeline2_0_1_0/1(d), pipeline2_0_1_2/1(d), pipeline2_1_1_0/1(d)
  pipeline0_2_1_2/1(q) -> cmult0_2_1/3
  c_to_ri2_1/2 -> pipeline0_2_1_3/1(d), pipeline1_1_1_3/1(d), pipeline2_0_1_1/1(d), pipeline2_0_1_3/1(d), pipeline2_1_1_1/1(d)
  pipeline0_2_1_3/1(q) -> cmult0_2_1/4
  cmult0_2_1/1 -> cvrt0_2_1_real/1(din)
  cmult0_2_1/2 -> cvrt0_2_1_imag/1(din)
  cvrt0_2_1_real/1(dout) -> ri_to_c0_2_1/1
  cvrt0_2_1_imag/1(dout) -> ri_to_c0_2_1/2
  ri_to_c0_2_1/1 -> pack0_2/2(in2)
  pack0_2/1(bus_out) -> din0_x_din2*/1
  pipeline0_3_0_0/1(q) -> cmult0_3_0/1
  pipeline0_3_0_1/1(q) -> cmult0_3_0/2
  c_to_ri3_0/1 -> pipeline0_3_0_2/1(d), pipeline1_2_0_2/1(d), pipeline2_1_0_2/1(d), pipeline3_0_0_0/1(d), pipeline3_0_0_2/1(d)
  pipeline0_3_0_2/1(q) -> cmult0_3_0/3
  c_to_ri3_0/2 -> pipeline0_3_0_3/1(d), pipeline1_2_0_3/1(d), pipeline2_1_0_3/1(d), pipeline3_0_0_1/1(d), pipeline3_0_0_3/1(d)
  pipeline0_3_0_3/1(q) -> cmult0_3_0/4
  cmult0_3_0/1 -> cvrt0_3_0_real/1(din)
  cmult0_3_0/2 -> cvrt0_3_0_imag/1(din)
  cvrt0_3_0_real/1(dout) -> ri_to_c0_3_0/1
  cvrt0_3_0_imag/1(dout) -> ri_to_c0_3_0/2
  ri_to_c0_3_0/1 -> pack0_3/1(in1)
  pipeline0_3_1_0/1(q) -> cmult0_3_1/1
  pipeline0_3_1_1/1(q) -> cmult0_3_1/2
  c_to_ri3_1/1 -> pipeline0_3_1_2/1(d), pipeline1_2_1_2/1(d), pipeline2_1_1_2/1(d), pipeline3_0_1_0/1(d), pipeline3_0_1_2/1(d)
  pipeline0_3_1_2/1(q) -> cmult0_3_1/3
  c_to_ri3_1/2 -> pipeline0_3_1_3/1(d), pipeline1_2_1_3/1(d), pipeline2_1_1_3/1(d), pipeline3_0_1_1/1(d), pipeline3_0_1_3/1(d)
  pipeline0_3_1_3/1(q) -> cmult0_3_1/4
  cmult0_3_1/1 -> cvrt0_3_1_real/1(din)
  cmult0_3_1/2 -> cvrt0_3_1_imag/1(din)
  cvrt0_3_1_real/1(dout) -> ri_to_c0_3_1/1
  cvrt0_3_1_imag/1(dout) -> ri_to_c0_3_1/2
  ri_to_c0_3_1/1 -> pack0_3/2(in2)
  pack0_3/1(bus_out) -> din0_x_din3*/1
  pipeline1_0_0_0/1(q) -> cmult1_0_0/1
  pipeline1_0_0_1/1(q) -> cmult1_0_0/2
  pipeline1_0_0_2/1(q) -> cmult1_0_0/3
  pipeline1_0_0_3/1(q) -> cmult1_0_0/4
  cmult1_0_0/1 -> cvrt1_0_0_real/1(din)
  cmult1_0_0/2 -> cvrt1_0_0_imag/1(din)
  cvrt1_0_0_real/1(dout) -> ri_to_c1_0_0/1
  cvrt1_0_0_imag/1(dout) -> ri_to_c1_0_0/2
  ri_to_c1_0_0/1 -> pack1_0/1(in1)
  pipeline1_0_1_0/1(q) -> cmult1_0_1/1
  pipeline1_0_1_1/1(q) -> cmult1_0_1/2
  pipeline1_0_1_2/1(q) -> cmult1_0_1/3
  pipeline1_0_1_3/1(q) -> cmult1_0_1/4
  cmult1_0_1/1 -> cvrt1_0_1_real/1(din)
  cmult1_0_1/2 -> cvrt1_0_1_imag/1(din)
  cvrt1_0_1_real/1(dout) -> ri_to_c1_0_1/1
  cvrt1_0_1_imag/1(dout) -> ri_to_c1_0_1/2
  ri_to_c1_0_1/1 -> pack1_0/2(in2)
  pack1_0/1(bus_out) -> din1_x_din1*/1
  pipeline1_1_0_0/1(q) -> cmult1_1_0/1
  pipeline1_1_0_1/1(q) -> cmult1_1_0/2
  pipeline1_1_0_2/1(q) -> cmult1_1_0/3
  pipeline1_1_0_3/1(q) -> cmult1_1_0/4
  cmult1_1_0/1 -> cvrt1_1_0_real/1(din)
  cmult1_1_0/2 -> cvrt1_1_0_imag/1(din)
  cvrt1_1_0_real/1(dout) -> ri_to_c1_1_0/1
  cvrt1_1_0_imag/1(dout) -> ri_to_c1_1_0/2
  ri_to_c1_1_0/1 -> pack1_1/1(in1)
  pipeline1_1_1_0/1(q) -> cmult1_1_1/1
  pipeline1_1_1_1/1(q) -> cmult1_1_1/2
  pipeline1_1_1_2/1(q) -> cmult1_1_1/3
  pipeline1_1_1_3/1(q) -> cmult1_1_1/4
  cmult1_1_1/1 -> cvrt1_1_1_real/1(din)
  cmult1_1_1/2 -> cvrt1_1_1_imag/1(din)
  cvrt1_1_1_real/1(dout) -> ri_to_c1_1_1/1
  cvrt1_1_1_imag/1(dout) -> ri_to_c1_1_1/2
  ri_to_c1_1_1/1 -> pack1_1/2(in2)
  pack1_1/1(bus_out) -> din1_x_din2*/1
  pipeline1_2_0_0/1(q) -> cmult1_2_0/1
  pipeline1_2_0_1/1(q) -> cmult1_2_0/2
  pipeline1_2_0_2/1(q) -> cmult1_2_0/3
  pipeline1_2_0_3/1(q) -> cmult1_2_0/4
  cmult1_2_0/1 -> cvrt1_2_0_real/1(din)
  cmult1_2_0/2 -> cvrt1_2_0_imag/1(din)
  cvrt1_2_0_real/1(dout) -> ri_to_c1_2_0/1
  cvrt1_2_0_imag/1(dout) -> ri_to_c1_2_0/2
  ri_to_c1_2_0/1 -> pack1_2/1(in1)
  pipeline1_2_1_0/1(q) -> cmult1_2_1/1
  pipeline1_2_1_1/1(q) -> cmult1_2_1/2
  pipeline1_2_1_2/1(q) -> cmult1_2_1/3
  pipeline1_2_1_3/1(q) -> cmult1_2_1/4
  cmult1_2_1/1 -> cvrt1_2_1_real/1(din)
  cmult1_2_1/2 -> cvrt1_2_1_imag/1(din)
  cvrt1_2_1_real/1(dout) -> ri_to_c1_2_1/1
  cvrt1_2_1_imag/1(dout) -> ri_to_c1_2_1/2
  ri_to_c1_2_1/1 -> pack1_2/2(in2)
  pack1_2/1(bus_out) -> din1_x_din3*/1
  pipeline2_0_0_0/1(q) -> cmult2_0_0/1
  pipeline2_0_0_1/1(q) -> cmult2_0_0/2
  pipeline2_0_0_2/1(q) -> cmult2_0_0/3
  pipeline2_0_0_3/1(q) -> cmult2_0_0/4
  cmult2_0_0/1 -> cvrt2_0_0_real/1(din)
  cmult2_0_0/2 -> cvrt2_0_0_imag/1(din)
  cvrt2_0_0_real/1(dout) -> ri_to_c2_0_0/1
  cvrt2_0_0_imag/1(dout) -> ri_to_c2_0_0/2
  ri_to_c2_0_0/1 -> pack2_0/1(in1)
  pipeline2_0_1_0/1(q) -> cmult2_0_1/1
  pipeline2_0_1_1/1(q) -> cmult2_0_1/2
  pipeline2_0_1_2/1(q) -> cmult2_0_1/3
  pipeline2_0_1_3/1(q) -> cmult2_0_1/4
  cmult2_0_1/1 -> cvrt2_0_1_real/1(din)
  cmult2_0_1/2 -> cvrt2_0_1_imag/1(din)
  cvrt2_0_1_real/1(dout) -> ri_to_c2_0_1/1
  cvrt2_0_1_imag/1(dout) -> ri_to_c2_0_1/2
  ri_to_c2_0_1/1 -> pack2_0/2(in2)
  pack2_0/1(bus_out) -> din2_x_din2*/1
  pipeline2_1_0_0/1(q) -> cmult2_1_0/1
  pipeline2_1_0_1/1(q) -> cmult2_1_0/2
  pipeline2_1_0_2/1(q) -> cmult2_1_0/3
  pipeline2_1_0_3/1(q) -> cmult2_1_0/4
  cmult2_1_0/1 -> cvrt2_1_0_real/1(din)
  cmult2_1_0/2 -> cvrt2_1_0_imag/1(din)
  cvrt2_1_0_real/1(dout) -> ri_to_c2_1_0/1
  cvrt2_1_0_imag/1(dout) -> ri_to_c2_1_0/2
  ri_to_c2_1_0/1 -> pack2_1/1(in1)
  pipeline2_1_1_0/1(q) -> cmult2_1_1/1
  pipeline2_1_1_1/1(q) -> cmult2_1_1/2
  pipeline2_1_1_2/1(q) -> cmult2_1_1/3
  pipeline2_1_1_3/1(q) -> cmult2_1_1/4
  cmult2_1_1/1 -> cvrt2_1_1_real/1(din)
  cmult2_1_1/2 -> cvrt2_1_1_imag/1(din)
  cvrt2_1_1_real/1(dout) -> ri_to_c2_1_1/1
  cvrt2_1_1_imag/1(dout) -> ri_to_c2_1_1/2
  ri_to_c2_1_1/1 -> pack2_1/2(in2)
  pack2_1/1(bus_out) -> din2_x_din3*/1
  pipeline3_0_0_0/1(q) -> cmult3_0_0/1
  pipeline3_0_0_1/1(q) -> cmult3_0_0/2
  pipeline3_0_0_2/1(q) -> cmult3_0_0/3
  pipeline3_0_0_3/1(q) -> cmult3_0_0/4
  cmult3_0_0/1 -> cvrt3_0_0_real/1(din)
  cmult3_0_0/2 -> cvrt3_0_0_imag/1(din)
  cvrt3_0_0_real/1(dout) -> ri_to_c3_0_0/1
  cvrt3_0_0_imag/1(dout) -> ri_to_c3_0_0/2
  ri_to_c3_0_0/1 -> pack3_0/1(in1)
  pipeline3_0_1_0/1(q) -> cmult3_0_1/1
  pipeline3_0_1_1/1(q) -> cmult3_0_1/2
  pipeline3_0_1_2/1(q) -> cmult3_0_1/3
  pipeline3_0_1_3/1(q) -> cmult3_0_1/4
  cmult3_0_1/1 -> cvrt3_0_1_real/1(din)
  cmult3_0_1/2 -> cvrt3_0_1_imag/1(din)
  cvrt3_0_1_real/1(dout) -> ri_to_c3_0_1/1
  cvrt3_0_1_imag/1(dout) -> ri_to_c3_0_1/2
  ri_to_c3_0_1/1 -> pack3_0/2(in2)
  pack3_0/1(bus_out) -> din3_x_din3*/1
